simulink model "run_sim_paper_scenario"  (R2020a)
settings: Solver=ode4  StartTime=0.0  StopTime=30.0  FixedStep=0.01  RelTol=1e-3
values from neighbouring files (symbols this model uses):
  alfa_theta = 20    [init_sim_paper_scenario.m]
  alfa_theta_obs = 100    [init_sim_paper_scenario.m]
  beta1 = 1.2    [init_sim_paper_scenario.m]
  beta2 = 0.8    [init_sim_paper_scenario.m]
  beta_Phi_1 = pp0 * cal_frac_squ( 3, p_p0_plus_1, q_p0_plus_1 )                          * cal_frac_squ( eps_s_bar / pi, p_p0_min_2, q_p0_min_2 )                          / ( 2 * ( 2 * pp0 - 1 ) * tanh( gamma0 * ( eps_s_bar / pi ) / 2 ) )                          - ( cal_frac_squ( 3, p_p0_plus_1, q_p0_plus_1 ) * gamma0 / ( 4 * ( 2 * pp0 -1 ) ) )                          * cal_frac_squ( eps_s_bar / pi, p_p0_min_ ...(+136 chars)    [init_sim_paper_scenario.m]
  beta_Phi_2 = ( 1 - pp0 ) * cal_frac_squ( 3, p_p0_plus_1, q_p0_plus_1 )                          / ( 2 * ( 1 - 2 * pp0 ) * cal_frac_squ( eps_s_bar / pi, p_p0_0, q_p0_0 ) * tanh( gamma0 * ( eps_s_bar / pi ) / 2 ) )                          - ( cal_frac_squ( 3, p_p0_plus_1, q_p0_plus_1 ) * gamma0 / ( 4 * ( 1 - 2 * pp0 ) ) )                          * cal_frac_squ( eps_s_bar / pi, p_1_min_p0, q_1_min_p0 )          ...(+112 chars)    [init_sim_paper_scenario.m]
  c1_diff_sigma_bar_v = diag([25; 30; 20])    [init_sim_paper_scenario.m]
  c1_diff_sigma_bar_w = diag([12; 12; 12])    [init_sim_paper_scenario.m]
  c1_diff_ui = diag([25; 30; 20])    [init_sim_paper_scenario.m]
  c1v = diag([5.8; 6.5; 6.5])    [init_sim_paper_scenario.m]
  c2_diff_sigma_bar_v = diag([50; 50; 10])    [init_sim_paper_scenario.m]
  c2_diff_sigma_bar_w = diag([12; 12; 12])    [init_sim_paper_scenario.m]
  c2_diff_ui = diag([50; 50; 10])    [init_sim_paper_scenario.m]
  c2v = diag([5.8; 6.5; 6.5])    [init_sim_paper_scenario.m]
  c3_diff_sigma_bar_v = diag([15; 15; 10])    [init_sim_paper_scenario.m]
  c3_diff_sigma_bar_w = diag([15; 15; 15])    [init_sim_paper_scenario.m]
  c3_diff_ui = diag([15; 15; 10])    [init_sim_paper_scenario.m]
  c3v = diag([4.8; 6.4; 6.0])    [init_sim_paper_scenario.m]
  c_w_1 = diag( [20; 15; 15] )    [init_sim_paper_scenario.m]
  c_w_2 = diag( [20; 15; 15] )    [init_sim_paper_scenario.m]
  c_w_3 = diag( [2; 2; 2] )    [init_sim_paper_scenario.m]
  cS0 = diag( [4.5; 4.5; 4.5] )    [init_sim_paper_scenario.m]
  delta_p_i_0 = zeros(3, NF)    [init_sim_paper_scenario.m]
  delta_v_i_0 = zeros(3, NF)    [init_sim_paper_scenario.m]
  dp_aa_t = 0.2 * ones(3, 5) + ( 1.0 - 0.2 ) * rand(3, 5)    [init_sim_paper_scenario.m]
  dp_ff_t = [ 0.4 * ones(1, 5) + ( 1.0 - 0.4 ) * rand(1, 5);                      0.4 * ones(1, 5) + ( 1.0 - 0.4 ) * rand(1, 5);                      0.2 * ones(1, 5) + ( 0.6 - 0.2 ) * rand(1, 5) ]    [init_sim_paper_scenario.m]
  dp_phi_t = ( - pi / 2 ) * ones(3, 5) + ( pi / 2 - ( - pi / 2 ) ) * rand(3, 5)    [init_sim_paper_scenario.m]
  dw_aa_t = 0.2 * ones(3, 5) + ( 1.0 - 0.2 ) * rand(3, 5)    [init_sim_paper_scenario.m]
  dw_ff_t = [ 0.4 * ones(1, 5) + ( 1.0 - 0.4 ) * rand(1, 5);                      0.4 * ones(1, 5) + ( 1.0 - 0.4 ) * rand(1, 5);                      0.2 * ones(1, 5) + ( 0.6 - 0.2 ) * rand(1, 5) ]    [init_sim_paper_scenario.m]
  dw_phi_t = ( - pi / 2 ) * ones(3, 5) + ( pi / 2 - ( - pi / 2 ) ) * rand(3, 5)    [init_sim_paper_scenario.m]
  dwci_init = zeros(3,5)    [init_sim_paper_scenario.m]
  eps_s_bar_div_pi = eps_s_bar / pi    (= 0.03)    [init_sim_paper_scenario.m]
  etai_0 = zeros(3,5)    [init_sim_paper_scenario.m]
  gamma0 = 20    [init_sim_paper_scenario.m]
  h1w = diag([20.0; 20.0; 20.0])    [init_sim_paper_scenario.m]
  h2w = diag([30.0; 35.0; 35.0])    [init_sim_paper_scenario.m]
  h3w = diag([30.0; 25.0; 30.0])    [init_sim_paper_scenario.m]
  Ji = zeros(3,3,NF)    [init_sim_paper_scenario.m]
  k_J_0 = diag( [1; 1; 1] )    [init_sim_paper_scenario.m]
  kai_1_t = 0.02    [init_sim_paper_scenario.m]
  kai_3_t = 0.1    [init_sim_paper_scenario.m]
  kai_chi_1 = diag([6; 6; 6])    [init_sim_paper_scenario.m]
  kai_chi_2 = diag([6; 6; 6])    [init_sim_paper_scenario.m]
  kai_u_1 = diag([8; 8; 8])    [init_sim_paper_scenario.m]
  kai_u_2 = diag([8; 8; 8])    [init_sim_paper_scenario.m]
  ksii_0 = zeros(3,5)    [init_sim_paper_scenario.m]
  l1v = diag([20; 20; 20])    [init_sim_paper_scenario.m]
  l2v = diag([30; 30; 30])    [init_sim_paper_scenario.m]
  Lamd_diff_sigma_bar_v = 0.5    [init_sim_paper_scenario.m]
  Lamd_diff_sigma_bar_w = 0.8    [init_sim_paper_scenario.m]
  Lamd_diff_ui = 0.8    [init_sim_paper_scenario.m]
  mass_i = zeros(1,NF)    [init_sim_paper_scenario.m]
  Mii = diag([1;0;0;0;1])    [init_sim_paper_scenario.m]
  mu_c_theta = 100    [init_sim_paper_scenario.m]
  mu_d_w = 100    [init_sim_paper_scenario.m]
  pos0 = zeros(3, 1)    [init_sim_paper_scenario.m]
  pp0 = 8 / 11    (= 0.727272727273)    [init_sim_paper_scenario.m]    (also in plot_sim_paper_scenario.m = plot3( ksi0(1, kkt), ksi0(2, kkt), ksi0(3, kkt),            )
  PZ0 = P0(3)    [init_sim_paper_scenario.m]
  PZ1 = 10    [init_sim_paper_scenario.m]
  Qci_init = repmat([1;0;0;0],1,NF)    [init_sim_paper_scenario.m]
  R0 = 4    [init_sim_paper_scenario.m]
  R1 = 8    [init_sim_paper_scenario.m]
  Rci_init = zeros(3,3,NF)    [init_sim_paper_scenario.m]
  Ri_init = zeros(3,3,NF)    [init_sim_paper_scenario.m]
  Rx2 = 10    [init_sim_paper_scenario.m]
  Ry2 = 6    [init_sim_paper_scenario.m]
  Rz2 = 4    [init_sim_paper_scenario.m]
  T0 = 0    [init_sim_paper_scenario.m]
  T1 = tseq1    (= 10)    [init_sim_paper_scenario.m]
  T12 = tseq1 + tseq12    (= 20)    [init_sim_paper_scenario.m]
  T2 = tseq1 + tseq12 + tseq2    (= 30)    [init_sim_paper_scenario.m]
  theta0 = ( 2 / 5 ) * pi    (= 1.25663706144)    [init_sim_paper_scenario.m]
  thr_p_plus_1 = cal_frac_squ( 3, p_p0_plus_1, q_p0_plus_1 )    [init_sim_paper_scenario.m]
  ui_init = zeros(3,NF)    [init_sim_paper_scenario.m]
  vel0 = zeros(3, 1)    [init_sim_paper_scenario.m]
  wci_init = zeros(3,5)    [init_sim_paper_scenario.m]
  Wij = [0,0,1,0,0;              0,0,1,1,0;              1,0,0,0,1;              0,1,1,0,0;              0,0,1,0,0]    [init_sim_paper_scenario.m]
  X1 = 8    [init_sim_paper_scenario.m]
  X2 = 2    [init_sim_paper_scenario.m]
  X3 = 3    [init_sim_paper_scenario.m]
  Y1 = 10    [init_sim_paper_scenario.m]
  Y2 = 2    [init_sim_paper_scenario.m]
  Y3 = 4    [init_sim_paper_scenario.m]
  Z1 = 4    [init_sim_paper_scenario.m]
  Z2 = -6    [init_sim_paper_scenario.m]
  Z3 = 2    [init_sim_paper_scenario.m]
  zeta_diff_sigma_bar_v = 0.08    [init_sim_paper_scenario.m]
  zeta_diff_sigma_bar_w = 0.3    [init_sim_paper_scenario.m]
  zeta_diff_ui = 0.05    [init_sim_paper_scenario.m]
undefined symbols (not defined in the file or in its folder): cal_frac_squ, p_2_p0, p_alfav1, p_alfav2, p_alfaw1, p_alfaw2, p_beta1, p_beta2, p_beta_w_1, p_beta_w_2, p_dbeta1, p_dbeta2, p_gamma1_pos, p_gamma1_vel, p_gamma2_pos, p_gamma2_vel, p_p0_min_1, p_p0_plus_1, q_2_p0, q_alfav1, q_alfav2, q_alfaw1, q_alfaw2, q_beta1, q_beta2, q_beta_w_1, q_beta_w_2, q_dbeta1, q_dbeta2, q_gamma1_pos, q_gamma1_vel, q_gamma2_pos, q_gamma2_vel, q_p0_min_1, q_p0_plus_1, Qei_init, Qi_init, Rei_init, V_Phi_Rei_init, wei_init, wi_init
(part 1 of 10)
settings Model: Creator=zzy  LastModifiedBy=Hershey.A
settings DataIOCC: ReturnWorkspaceOutputs=off
settings DebuggingCC: ArithmeticOperatorsInVariantConditions=warning
settings SFSimCC: SimUseLocalCustomCode=off  CustomCodeUndefinedFunction=UseInterfaceOnly
settings RTWCC: RTWUseLocalCustomCode=off

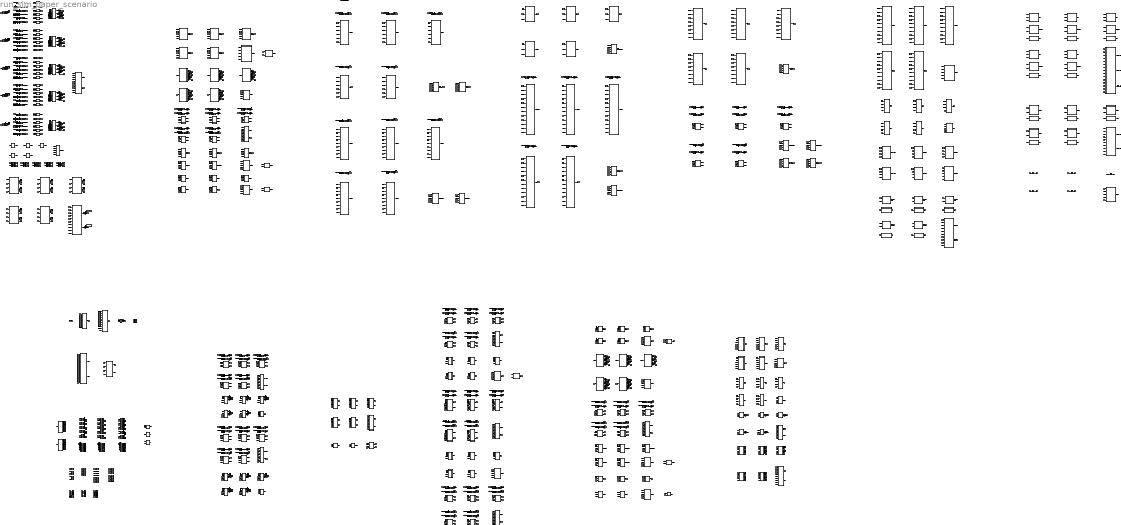
== system run_sim_paper_scenario ==
  Abs{,1..29} (30 alike) : Abs
  Add{,1..12,14,16..18,20..22,24..26,28..29} (25 alike) : Sum
  Add{13,15,19,23,27} (5 alike) : Sum  Inputs=+-
  Clock : Clock
  Constant : Constant  Value=T1
  Constant{1,4,9,19,24,149,154,159,164,169} (10 alike) : Constant  Value=q_beta1
  Constant{5,10,14,16,20,39,46,54,61,79,101,103,108,113,118,148,153,158,163,168} (20 alike) : Constant  Value=alfa_theta
  Constant{100,102,107,112,117} (5 alike) : Constant  Value=p_alfav1
  Constant{97,104,109,114,119} (5 alike) : Constant  Value=q_alfav1
  Constant{98,105,110,115,120} (5 alike) : Constant  Value=p_alfav2
  Constant{99,106,111,116,121} (5 alike) : Constant  Value=q_alfav2
  Constant{2,6,11,15,21,150,155,160,165,170} (10 alike) : Constant  Value=p_beta2
  Constant{3,7,12,17,22,151,156,161,166,171} (10 alike) : Constant  Value=q_beta2
  Constant{122,124,126,128,140} (5 alike) : Constant  Value=c1v
  Constant{123,125,127,139,141} (5 alike) : Constant  Value=c2v
  Constant129 : Constant  Value=R0
  Constant{8,13,18,23,63,147,152,157,162,167} (10 alike) : Constant  Value=p_beta1
  Constant130 : Constant  Value=R1
  Constant131 : Constant  Value=T0
  Constant132 : Constant  Value=Rz2
  Constant133 : Constant  Value=Ry2
  Constant134 : Constant  Value=Rx2
  Constant135 : Constant  Value=X1
  Constant136 : Constant  Value=X2
  Constant137 : Constant  Value=Y1
  Constant138 : Constant  Value=Y2
  Constant{92..96,142..146} (10 alike) : Constant  Value=c3v
  Constant{172,174,176,178,180} (5 alike) : Constant  Value=kai_u_1
  Constant{173,175,177,179,181} (5 alike) : Constant  Value=kai_u_2
  Constant{182..183,189,199,202,205,209,212,219,252} (10 alike) : Constant  Value=l2v
  Constant{184..186,193..196,198,283..284} (10 alike) : Constant  Value=alfa_theta_obs
  Constant{187,190,197,200,203,206,210,213,230,263} (10 alike) : Constant  Value=l1v
  Constant188 : Constant  Value=delta_p_i_0(:,4)
  Constant191 : Constant  Value=mass_i
  Constant192 : Constant  Value=delta_p_i_0(:,5)
  Constant201 : Constant  Value=delta_v_i_0(:,1)
  Constant204 : Constant  Value=delta_v_i_0(:,2)
  Constant207 : Constant  Value=delta_v_i_0(:,3)
  Constant208 : Constant  Value=delta_p_i_0(:,1)
  Constant211 : Constant  Value=delta_v_i_0(:,4)
  Constant214 : Constant  Value=delta_v_i_0(:,5)
  Constant{215,220,270,275,279} (5 alike) : Constant  Value=p_gamma1_pos
  Constant{216,267,271,276,280} (5 alike) : Constant  Value=q_gamma1_pos
  Constant{217,268,272,277,281} (5 alike) : Constant  Value=p_gamma2_pos
  Constant{218,269,273,278,282} (5 alike) : Constant  Value=q_gamma2_pos
  Constant221 : Constant  Value=Z1
  Constant222 : Constant  Value=Z2
  Constant{223,227,232,236,240} (5 alike) : Constant  Value=Wij
  Constant{224,228,233,237,242} (5 alike) : Constant  Value=Mii
  Constant225 : Constant  Value=theta0
  Constant226 : Constant  Value=Z3
  Constant229 : Constant  Value=Y3
  Constant231 : Constant  Value=kai_1_t
  Constant234 : Constant  Value=X3
  Constant235 : Constant  Value=kai_3_t
  Constant238 : Constant  Value=T1
  Constant239 : Constant  Value=T12
  Constant241 : Constant  Value=delta_p_i_0(:,2)
  Constant{243,286,289,292,295} (5 alike) : Constant  Value=dp_phi_t
  Constant{244,287,290,293,296} (5 alike) : Constant  Value=dp_ff_t
  Constant{245,249,254,258,262} (5 alike) : Constant  Value=p_gamma1_vel
  Constant{246,250,255,259,264} (5 alike) : Constant  Value=q_gamma1_vel
  Constant{247,251,256,260,265} (5 alike) : Constant  Value=p_gamma2_vel
  Constant{248,253,257,261,266} (5 alike) : Constant  Value=q_gamma2_vel
  Constant{25,27,29,31,33,82,84,86,88,90} (10 alike) : Constant  Value=kai_chi_2
  Constant{26,28,30,32,34,83,85,87,89,91} (10 alike) : Constant  Value=kai_chi_1
  Constant274 : Constant  Value=delta_p_i_0(:,3)
  Constant{285,288,291,294,297} (5 alike) : Constant  Value=dp_aa_t
  Constant{298,331,362,619,639} (5 alike) : Constant  Value=0
  Constant{299,411,488,556,621} (5 alike) : Constant  Value=p_p0_plus_1
  Constant{300,355,433,510,521} (5 alike) : Constant  Value=p_2_p0
  Constant{301,306,308,310,316,321,324,326,343,347,352,354,357,363,590,593,598,601,603,620,624,629,631,634,640} (25 alike) : Constant
  Constant{302,309,312..313,317,325,327..328,345..346,348,356,358..359,364..365,591..592,594,602,615..616,622..623,625,633,635..636,641..642} (30 alike) : Constant  Value=3
  Constant{303,314,318,329,349,360,595,617,626,637} (10 alike) : Constant  Value=2
  Constant{304,319,350,596,627} (5 alike) : Constant  Value=c1_diff_ui
  Constant{305,320,351,597,628} (5 alike) : Constant  Value=c2_diff_ui
  Constant{307,323,353,600,630} (5 alike) : Constant  Value=c3_diff_ui
  Constant{311,366,444,522,577} (5 alike) : Constant  Value=q_2_p0
  Constant{315,330,361,618,638} (5 alike) : Constant  Value=Lamd_diff_ui
  Constant{322,377,455,483,485,487,490,492,533,588,609,611..614} (15 alike) : Constant  Value=cS0
  Constant{332,335,337,339,341} (5 alike) : Constant  Value=p_p0_min_1
  Constant{333,388,393,461,466,468,474,481,544..545,578,583,589,599,607} (15 alike) : Constant  Value=gamma0
  Constant{334,336,338,340,342} (5 alike) : Constant  Value=q_p0_min_1
  Constant{344,392,398..399,467,473,477,480,547,555,575,581,586,605,610} (15 alike) : Constant  Value=thr_p_plus_1
  Constant{35,42,49,57,75} (5 alike) : Constant  Value=q_dbeta1
  Constant{36,43,50,58,76} (5 alike) : Constant  Value=p_dbeta2
  Constant{367..376,378..382} (15 alike) : Constant  Value=zeta_diff_ui
  Constant{37,44,52,59,77} (5 alike) : Constant  Value=q_dbeta2
  Constant{38,45,53,60,78} (5 alike) : Constant  Value=p_dbeta1
  Constant{383..387,401,413,437,447,450..452,454,457,459,484,486,489,491,493,526,530,535,539,543} (25 alike) : Constant  Value=Ji
  Constant{389,395,463,470,476} (5 alike) : Constant  Value=pp0
  Constant{390,396,464,471,478,571,579,584,604,608} (10 alike) : Constant  Value=beta_Phi_1
  Constant{391,397,465,472,479,548..549,574,580,585} (10 alike) : Constant  Value=beta_Phi_2
  Constant{394,462,469,475,482,546,576,582,587,606} (10 alike) : Constant  Value=eps_s_bar_div_pi
  Constant{40,47,55,62,80} (5 alike) : Constant  Value=beta1
  Constant{400,425,445..446,448..449,453,456,458,460} (10 alike) : Constant  Value=h3w
  Constant{402,404,409,417,423} (5 alike) : Constant  Value=p_alfaw1
  Constant{403,405,412,418,424} (5 alike) : Constant  Value=mu_d_w
  Constant{406,414,419,426,429} (5 alike) : Constant  Value=q_alfaw1
  Constant{407,415,420,427,430} (5 alike) : Constant  Value=p_alfaw2
  Constant{408,416,421,428,431} (5 alike) : Constant  Value=q_alfaw2
  Constant{41,48,56,74,81} (5 alike) : Constant  Value=beta2
  Constant{410,422,499,560,632} (5 alike) : Constant  Value=q_p0_plus_1
  Constant{432,435,438,440,442} (5 alike) : Constant  Value=h1w
  Constant{434,436,439,441,443} (5 alike) : Constant  Value=h2w
  Constant{494,500,505,511,516} (5 alike) : Constant  Value=p_beta_w_1
  Constant{495,501,506,512,517} (5 alike) : Constant  Value=q_beta_w_1
  Constant{496,502,507,513,518} (5 alike) : Constant  Value=p_beta_w_2
  Constant{497,503,508,514,519} (5 alike) : Constant  Value=q_beta_w_2
  Constant{498,504,509,515,520} (5 alike) : Constant  Value=mu_c_theta
  Constant51 : Constant  Value=Qci_init
  Constant{523,527,531,536,540} (5 alike) : Constant  Value=c_w_1
  Constant{524,528,532,537,541} (5 alike) : Constant  Value=c_w_2
  Constant{525,529,534,538,542} (5 alike) : Constant  Value=c_w_3
  Constant{550..554} (5 alike) : Constant  Value=k_J_0
  Constant{557,561,564,567,570} (5 alike) : Constant  Value=dw_aa_t
  Constant{558,562,565,568,572} (5 alike) : Constant  Value=dw_ff_t
  Constant{559,563,566,569,573} (5 alike) : Constant  Value=dw_phi_t
  Constant64 : Constant  Value=T2
  Constant65 : Constant  Value=R0
  Constant66 : Constant  Value=R1
  Constant67 : Constant  Value=Rx2
  Constant68 : Constant  Value=Ry2
  Constant69 : Constant  Value=Rz2
  Constant70 : Constant  Value=T2
  Constant71 : Constant  Value=T1
  Constant72 : Constant  Value=PZ0
  Constant73 : Constant  Value=PZ1
  Demux{,1..141} (142 alike) : Demux  Outputs=3
  Display{1..5,7..21,26..63,69..172} (162 alike) : Display
  Integrator{1..15,46..50} (20 alike) : Integrator  InitialCondition=zeros(3,1)
  Integrator17 : Integrator  InitialCondition=V_Phi_Rei_init(:,2)
  Integrator19 : Integrator  InitialCondition=V_Phi_Rei_init(:,3)
  Integrator20 : Integrator  InitialCondition=V_Phi_Rei_init(:,1)
  Integrator21 : Integrator  InitialCondition=wi_init(:,1)
  Integrator22 : Integrator  InitialCondition=wi_init(:,2)
  Integrator23 : Integrator  InitialCondition=wi_init(:,3)
  Integrator24 : Integrator  InitialCondition=wi_init(:,4)
  Integrator25 : Integrator  InitialCondition=wi_init(:,5)
  Integrator26 : Integrator  InitialCondition=Qi_init(:,1)
  Integrator27 : Integrator  InitialCondition=Qi_init(:,2)
  Integrator28 : Integrator  InitialCondition=Qi_init(:,3)
  Integrator29 : Integrator  InitialCondition=Qi_init(:,4)
  Integrator30 : Integrator  InitialCondition=Qi_init(:,5)
  Integrator31 : Integrator  InitialCondition=Qei_init(:,1)
  Integrator32 : Integrator  InitialCondition=Qei_init(:,2)
  Integrator33 : Integrator  InitialCondition=Qei_init(:,3)
  Integrator34 : Integrator  InitialCondition=Qei_init(:,4)
  Integrator35 : Integrator  InitialCondition=Qei_init(:,5)
  Integrator42 : Integrator  InitialCondition=V_Phi_Rei_init(:,4)
  Integrator44 : Integrator  InitialCondition=V_Phi_Rei_init(:,5)
  Interpreted MATLAB Function{,1..124} (125 alike) : MATLABFcn  MATLABFcn=cal_frac_squ(u(1:3),u(4),u(5))
  Memory : Memory  InitialCondition=ui_init
  Memory1 : Memory  InitialCondition=etai_0
  Memory{9..11,13,18..25} (12 alike) : Memory  InitialCondition=zeros(3,5)
  Memory12 : Memory  InitialCondition=V_Phi_Rei_init
  Memory14 : Memory  InitialCondition=wci_init
  Memory15 : Memory  InitialCondition=dwci_init
  Memory16 : Memory  InitialCondition=Qci_init
  Memory17 : Memory  InitialCondition=Rci_init
  Memory2 : Memory  InitialCondition=ksii_0
  Memory3 : Memory  InitialCondition=Qi_init
  Memory4 : Memory  InitialCondition=Ri_init
  Memory5 : Memory  InitialCondition=wi_init
  Memory6 : Memory  InitialCondition=wei_init
  Memory7 : Memory  InitialCondition=Qei_init
  Memory8 : Memory  InitialCondition=Rei_init
  Mux{1..40,109..118,120..129,136..170,180,187..215} (125 alike) : Mux  Inputs=3
  Mux{41..108,119,130..135,171..179,181..186} (90 alike) : Mux  Inputs=2
  Product{,1..9} (10 alike) : Product
  Qei dynam agent 1 : MATLAB Function  TreatAsAtomicUnit=on
  Qei dynam agent 2 : MATLAB Function  TreatAsAtomicUnit=on
  Qei dynam agent 3 : MATLAB Function  TreatAsAtomicUnit=on
  Qei dynam agent 4 : MATLAB Function  TreatAsAtomicUnit=on
  Qei dynam agent 5 : MATLAB Function  TreatAsAtomicUnit=on
  Qi dynam agent 1 : MATLAB Function  TreatAsAtomicUnit=on
  Qi dynam agent 2 : MATLAB Function  TreatAsAtomicUnit=on
  Qi dynam agent 3 : MATLAB Function  TreatAsAtomicUnit=on
  Qi dynam agent 4 : MATLAB Function  TreatAsAtomicUnit=on
  Qi dynam agent 5 : MATLAB Function  TreatAsAtomicUnit=on
  Scope{1..2,13..15} (5 alike) : Scope  NumInputPorts=3
  Step : Step  Time=T1+0.01  SampleTime=0
  To Workspace : ToWorkspace  VariableName=eta_d_est_vec  SampleTime=-1
  To Workspace1 : ToWorkspace  VariableName=dp_hat_vec  SampleTime=-1
  To Workspace10 : ToWorkspace  VariableName=eta_track_err_vec  SampleTime=-1
  To Workspace11 : ToWorkspace  VariableName=sigma_bar_v_hat_vec  SampleTime=-1
  To Workspace12 : ToWorkspace  VariableName=sigma_bar_v_vec  SampleTime=-1
  To Workspace13 : ToWorkspace  VariableName=sigma_bar_v_tilt_vec  SampleTime=-1
  To Workspace14 : ToWorkspace  VariableName=ui_vec  SampleTime=-1
  To Workspace15 : ToWorkspace  VariableName=chi_vec  SampleTime=-1
  To Workspace16 : ToWorkspace  VariableName=phi_vec  SampleTime=-1
  To Workspace17 : ToWorkspace  VariableName=ksi_est_err  SampleTime=-1
  To Workspace18 : ToWorkspace  VariableName=ksi_d_est_vec  SampleTime=-1
  To Workspace19 : ToWorkspace  VariableName=sigma_v_vec  SampleTime=-1
  To Workspace2 : ToWorkspace  VariableName=dp_vec  SampleTime=-1
  To Workspace20 : ToWorkspace  VariableName=delta_ksi_vec  SampleTime=-1
  To Workspace21 : ToWorkspace  VariableName=delta_eta_vec  SampleTime=-1
  To Workspace22 : ToWorkspace  VariableName=eta_est_err  SampleTime=-1
  To Workspace23 : ToWorkspace  VariableName=wci  SampleTime=-1
  To Workspace24 : ToWorkspace  VariableName=V_Phi_Rei  SampleTime=-1
  To Workspace25 : ToWorkspace  VariableName=dwi_tilt  SampleTime=-1
  To Workspace26 : ToWorkspace  VariableName=Qci  SampleTime=-1
  To Workspace27 : ToWorkspace  VariableName=sigma_bar_w_hat  SampleTime=-1
  To Workspace28 : ToWorkspace  VariableName=wei  SampleTime=-1
  To Workspace29 : ToWorkspace  VariableName=sigma_w  SampleTime=-1
  To Workspace3 : ToWorkspace  VariableName=u0  SampleTime=-1
  To Workspace30 : ToWorkspace  VariableName=sigma_bar_w  SampleTime=-1
  To Workspace31 : ToWorkspace  VariableName=Phi_psi_e  SampleTime=-1
  To Workspace32 : ToWorkspace  VariableName=Phi_bar_psi_e  SampleTime=-1
  To Workspace33 : ToWorkspace  VariableName=Qei  SampleTime=-1
  To Workspace34 : ToWorkspace  VariableName=wi  SampleTime=-1
  To Workspace35 : ToWorkspace  VariableName=Qi  SampleTime=-1
  To Workspace36 : ToWorkspace  VariableName=S_bar  SampleTime=-1
  To Workspace37 : ToWorkspace  VariableName=Si  SampleTime=-1
  To Workspace38 : ToWorkspace  VariableName=dwi  SampleTime=-1
  To Workspace39 : ToWorkspace  VariableName=dwi_hat  SampleTime=-1
  To Workspace4 : ToWorkspace  VariableName=eta0  SampleTime=-1
  To Workspace5 : ToWorkspace  VariableName=ksi0  SampleTime=-1
  To Workspace6 : ToWorkspace  VariableName=dp_tilt_vec  SampleTime=-1
  To Workspace7 : ToWorkspace  VariableName=eta_i_vec  SampleTime=-1
  To Workspace8 : ToWorkspace  VariableName=ksi_i_vec  SampleTime=-1
  To Workspace9 : ToWorkspace  VariableName=ksi_track_err_vec  SampleTime=-1
  cal Fi_S agent 1 : MATLAB Function  TreatAsAtomicUnit=on
  cal Fi_S agent 2 : MATLAB Function  TreatAsAtomicUnit=on
  cal Fi_S agent 3 : MATLAB Function  TreatAsAtomicUnit=on
  cal Fi_S agent 4 : MATLAB Function  TreatAsAtomicUnit=on
  cal Fi_S agent 5 : MATLAB Function  TreatAsAtomicUnit=on
  cal Phi_bar_psi_e agent 1 : MATLAB Function  TreatAsAtomicUnit=on
  cal Phi_bar_psi_e agent 2 : MATLAB Function  TreatAsAtomicUnit=on
  cal Phi_bar_psi_e agent 3 : MATLAB Function  TreatAsAtomicUnit=on
  cal Phi_bar_psi_e agent 4 : MATLAB Function  TreatAsAtomicUnit=on
  cal Phi_bar_psi_e agent 5 : MATLAB Function  TreatAsAtomicUnit=on
  cal Phi_psi_e agent 1 : MATLAB Function  TreatAsAtomicUnit=on
  cal Phi_psi_e agent 2 : MATLAB Function  TreatAsAtomicUnit=on
  cal Phi_psi_e agent 3 : MATLAB Function  TreatAsAtomicUnit=on
  cal Phi_psi_e agent 4 : MATLAB Function  TreatAsAtomicUnit=on
  cal Phi_psi_e agent 5 : MATLAB Function  TreatAsAtomicUnit=on
  cal Qci agent 1 : MATLAB Function  TreatAsAtomicUnit=on
  cal Qci agent 2 : MATLAB Function  TreatAsAtomicUnit=on
  cal Qci agent 3 : MATLAB Function  TreatAsAtomicUnit=on
  cal Qci agent 4 : MATLAB Function  TreatAsAtomicUnit=on
  cal Qci agent 5 : MATLAB Function  TreatAsAtomicUnit=on
  cal Rci agent 1 : MATLAB Function  TreatAsAtomicUnit=on
  cal Rci agent 2 : MATLAB Function  TreatAsAtomicUnit=on
  cal Rci agent 3 : MATLAB Function  TreatAsAtomicUnit=on
  cal Rci agent 4 : MATLAB Function  TreatAsAtomicUnit=on
  cal Rci agent 5 : MATLAB Function  TreatAsAtomicUnit=on
  cal Rci from ui : MATLAB Function  TreatAsAtomicUnit=on
  cal Rei : MATLAB Function  TreatAsAtomicUnit=on
  cal Rei agent 1 : MATLAB Function  TreatAsAtomicUnit=on
  cal Rei agent 2 : MATLAB Function  TreatAsAtomicUnit=on
  cal Rei agent 3 : MATLAB Function  TreatAsAtomicUnit=on
  cal Rei agent 4 : MATLAB Function  TreatAsAtomicUnit=on
  cal Rei agent 5 : MATLAB Function  TreatAsAtomicUnit=on
  cal Ri : MATLAB Function  TreatAsAtomicUnit=on
  cal Ri agent 1 : MATLAB Function  TreatAsAtomicUnit=on
  cal Ri agent 2 : MATLAB Function  TreatAsAtomicUnit=on
  cal Ri agent 3 : MATLAB Function  TreatAsAtomicUnit=on
  cal Ri agent 4 : MATLAB Function  TreatAsAtomicUnit=on
  cal Ri agent 5 : MATLAB Function  TreatAsAtomicUnit=on
  cal S_bar agent 1 : MATLAB Function  TreatAsAtomicUnit=on
  cal S_bar agent 2 : MATLAB Function  TreatAsAtomicUnit=on
  cal S_bar agent 3 : MATLAB Function  TreatAsAtomicUnit=on
  cal S_bar agent 4 : MATLAB Function  TreatAsAtomicUnit=on
  cal S_bar agent 5 : MATLAB Function  TreatAsAtomicUnit=on
  cal Si agent 1 : MATLAB Function  TreatAsAtomicUnit=on
  cal Si agent 2 : MATLAB Function  TreatAsAtomicUnit=on
  cal Si agent 3 : MATLAB Function  TreatAsAtomicUnit=on
  cal Si agent 4 : MATLAB Function  TreatAsAtomicUnit=on
  cal Si agent 5 : MATLAB Function  TreatAsAtomicUnit=on
  cal abs 1 : MATLAB Function  TreatAsAtomicUnit=on
  cal abs 10 : MATLAB Function  TreatAsAtomicUnit=on
  cal abs 11 : MATLAB Function  TreatAsAtomicUnit=on
  cal abs 12 : MATLAB Function  TreatAsAtomicUnit=on
  cal abs 13 : MATLAB Function  TreatAsAtomicUnit=on
  cal abs 14 : MATLAB Function  TreatAsAtomicUnit=on
  cal abs 15 : MATLAB Function  TreatAsAtomicUnit=on
  cal abs 16 : MATLAB Function  TreatAsAtomicUnit=on
  cal abs 17 : MATLAB Function  TreatAsAtomicUnit=on
  cal abs 18 : MATLAB Function  TreatAsAtomicUnit=on
  cal abs 19 : MATLAB Function  TreatAsAtomicUnit=on
  cal abs 2 : MATLAB Function  TreatAsAtomicUnit=on
  cal abs 20 : MATLAB Function  TreatAsAtomicUnit=on
  cal abs 21 : MATLAB Function  TreatAsAtomicUnit=on
  cal abs 22 : MATLAB Function  TreatAsAtomicUnit=on
  cal abs 23 : MATLAB Function  TreatAsAtomicUnit=on
  cal abs 24 : MATLAB Function  TreatAsAtomicUnit=on
  cal abs 25 : MATLAB Function  TreatAsAtomicUnit=on
  cal abs 26 : MATLAB Function  TreatAsAtomicUnit=on
  cal abs 27 : MATLAB Function  TreatAsAtomicUnit=on
  cal abs 28 : MATLAB Function  TreatAsAtomicUnit=on
  cal abs 29 : MATLAB Function  TreatAsAtomicUnit=on
  cal abs 3 : MATLAB Function  TreatAsAtomicUnit=on
  cal abs 30 : MATLAB Function  TreatAsAtomicUnit=on
  cal abs 31 : MATLAB Function  TreatAsAtomicUnit=on
  cal abs 32 : MATLAB Function  TreatAsAtomicUnit=on
  cal abs 33 : MATLAB Function  TreatAsAtomicUnit=on
  cal abs 34 : MATLAB Function  TreatAsAtomicUnit=on
  cal abs 35 : MATLAB Function  TreatAsAtomicUnit=on
  cal abs 36 : MATLAB Function  TreatAsAtomicUnit=on
  cal abs 37 : MATLAB Function  TreatAsAtomicUnit=on
  cal abs 38 : MATLAB Function  TreatAsAtomicUnit=on
  cal abs 39 : MATLAB Function  TreatAsAtomicUnit=on
  cal abs 4 : MATLAB Function  TreatAsAtomicUnit=on
  cal abs 40 : MATLAB Function  TreatAsAtomicUnit=on
  cal abs 41 : MATLAB Function  TreatAsAtomicUnit=on
  cal abs 42 : MATLAB Function  TreatAsAtomicUnit=on
  cal abs 43 : MATLAB Function  TreatAsAtomicUnit=on
  cal abs 44 : MATLAB Function  TreatAsAtomicUnit=on
  cal abs 45 : MATLAB Function  TreatAsAtomicUnit=on
  cal abs 46 : MATLAB Function  TreatAsAtomicUnit=on
  cal abs 47 : MATLAB Function  TreatAsAtomicUnit=on
  cal abs 48 : MATLAB Function  TreatAsAtomicUnit=on
  cal abs 49 : MATLAB Function  TreatAsAtomicUnit=on
  cal abs 5 : MATLAB Function  TreatAsAtomicUnit=on
  cal abs 50 : MATLAB Function  TreatAsAtomicUnit=on
  cal abs 51 : MATLAB Function  TreatAsAtomicUnit=on
  cal abs 52 : MATLAB Function  TreatAsAtomicUnit=on
  cal abs 53 : MATLAB Function  TreatAsAtomicUnit=on
  cal abs 54 : MATLAB Function  TreatAsAtomicUnit=on
  cal abs 55 : MATLAB Function  TreatAsAtomicUnit=on
  cal abs 56 : MATLAB Function  TreatAsAtomicUnit=on
  cal abs 57 : MATLAB Function  TreatAsAtomicUnit=on
  cal abs 58 : MATLAB Function  TreatAsAtomicUnit=on
  cal abs 59 : MATLAB Function  TreatAsAtomicUnit=on
  cal abs 6 : MATLAB Function  TreatAsAtomicUnit=on
  cal abs 60 : MATLAB Function  TreatAsAtomicUnit=on
  cal abs 61 : MATLAB Function  TreatAsAtomicUnit=on
  cal abs 62 : MATLAB Function  TreatAsAtomicUnit=on
  cal abs 63 : MATLAB Function  TreatAsAtomicUnit=on
  cal abs 64 : MATLAB Function  TreatAsAtomicUnit=on
  cal abs 65 : MATLAB Function  TreatAsAtomicUnit=on
  cal abs 66 : MATLAB Function  TreatAsAtomicUnit=on
  cal abs 67 : MATLAB Function  TreatAsAtomicUnit=on
  cal abs 68 : MATLAB Function  TreatAsAtomicUnit=on
  cal abs 69 : MATLAB Function  TreatAsAtomicUnit=on
  cal abs 7 : MATLAB Function  TreatAsAtomicUnit=on
  cal abs 70 : MATLAB Function  TreatAsAtomicUnit=on
  cal abs 71 : MATLAB Function  TreatAsAtomicUnit=on
  cal abs 72 : MATLAB Function  TreatAsAtomicUnit=on
  cal abs 73 : MATLAB Function  TreatAsAtomicUnit=on
  cal abs 74 : MATLAB Function  TreatAsAtomicUnit=on
  cal abs 75 : MATLAB Function  TreatAsAtomicUnit=on
  cal abs 76 : MATLAB Function  TreatAsAtomicUnit=on
  cal abs 77 : MATLAB Function  TreatAsAtomicUnit=on
  cal abs 78 : MATLAB Function  TreatAsAtomicUnit=on
  cal abs 79 : MATLAB Function  TreatAsAtomicUnit=on
  cal abs 8 : MATLAB Function  TreatAsAtomicUnit=on
  cal abs 80 : MATLAB Function  TreatAsAtomicUnit=on
  cal abs 81 : MATLAB Function  TreatAsAtomicUnit=on
  cal abs 82 : MATLAB Function  TreatAsAtomicUnit=on
  cal abs 83 : MATLAB Function  TreatAsAtomicUnit=on
  cal abs 84 : MATLAB Function  TreatAsAtomicUnit=on
  cal abs 85 : MATLAB Function  TreatAsAtomicUnit=on
  cal abs 86 : MATLAB Function  TreatAsAtomicUnit=on
  cal abs 87 : MATLAB Function  TreatAsAtomicUnit=on
  cal abs 88 : MATLAB Function  TreatAsAtomicUnit=on
  cal abs 89 : MATLAB Function  TreatAsAtomicUnit=on
  cal abs 9 : MATLAB Function  TreatAsAtomicUnit=on
  cal abs 90 : MATLAB Function  TreatAsAtomicUnit=on
  cal abs 91 : MATLAB Function  TreatAsAtomicUnit=on
  cal abs 92 : MATLAB Function  TreatAsAtomicUnit=on
  cal abs 93 : MATLAB Function  TreatAsAtomicUnit=on
  cal abs 94 : MATLAB Function  TreatAsAtomicUnit=on
  cal abs 95 : MATLAB Function  TreatAsAtomicUnit=on
  cal combine sigma_bar_v : MATLAB Function  TreatAsAtomicUnit=on
  cal combine sigma_bar_v_tilt : MATLAB Function  TreatAsAtomicUnit=on
  cal combine sigma_bar_w_tilt : MATLAB Function  TreatAsAtomicUnit=on
  cal d_sigma_w agent 1 : MATLAB Function  TreatAsAtomicUnit=on
  cal d_sigma_w agent 2 : MATLAB Function  TreatAsAtomicUnit=on
  cal d_sigma_w agent 3 : MATLAB Function  TreatAsAtomicUnit=on
  cal d_sigma_w agent 4 : MATLAB Function  TreatAsAtomicUnit=on
  cal d_sigma_w agent 5 : MATLAB Function  TreatAsAtomicUnit=on
  cal d_theta_err_ksi agent 1 : MATLAB Function  TreatAsAtomicUnit=on
  cal d_theta_err_ksi agent 2 : MATLAB Function  TreatAsAtomicUnit=on
  cal d_theta_err_ksi agent 3 : MATLAB Function  TreatAsAtomicUnit=on
  cal d_theta_err_ksi agent 4 : MATLAB Function  TreatAsAtomicUnit=on
  cal d_theta_err_ksi agent 5 : MATLAB Function  TreatAsAtomicUnit=on
  cal dchi agent 1 : MATLAB Function  TreatAsAtomicUnit=on
  cal dchi agent 2 : MATLAB Function  TreatAsAtomicUnit=on
  cal dchi agent 3 : MATLAB Function  TreatAsAtomicUnit=on
  cal dchi agent 4 : MATLAB Function  TreatAsAtomicUnit=on
  cal dchi agent 5 : MATLAB Function  TreatAsAtomicUnit=on
  cal differentiator d_sigma_bar_v_hat agent 1 : Subsystem
  cal differentiator d_sigma_bar_v_hat agent 2 : Subsystem
  cal differentiator d_sigma_bar_v_hat agent 3 : Subsystem
  cal differentiator d_sigma_bar_v_hat agent 4 : Subsystem
  cal differentiator d_sigma_bar_v_hat agent 5 : Subsystem
  cal differentiator d_sigma_bar_w_hat agent 1 : Subsystem
  cal differentiator d_sigma_bar_w_hat agent 2 : Subsystem
  cal differentiator d_sigma_bar_w_hat agent 3 : Subsystem
  cal differentiator d_sigma_bar_w_hat agent 4 : Subsystem
  cal differentiator d_sigma_bar_w_hat agent 5 : Subsystem
  cal disturbance observation error dp_tilt : MATLAB Function  TreatAsAtomicUnit=on
  cal divide pi : MATLAB Function  TreatAsAtomicUnit=on
  cal dp_hat agent 1 : MATLAB Function  TreatAsAtomicUnit=on
  cal dp_hat agent 2 : MATLAB Function  TreatAsAtomicUnit=on
  cal dp_hat agent 3 : MATLAB Function  TreatAsAtomicUnit=on
  cal dp_hat agent 4 : MATLAB Function  TreatAsAtomicUnit=on
  cal dp_hat agent 5 : MATLAB Function  TreatAsAtomicUnit=on
  cal duihat d2uihat by high-order differentiator node 1 : MATLAB Function  TreatAsAtomicUnit=on
  cal duihat d2uihat by high-order differentiator node 2 : MATLAB Function  TreatAsAtomicUnit=on
  cal duihat d2uihat by high-order differentiator node 3 : MATLAB Function  TreatAsAtomicUnit=on
  cal duihat d2uihat by high-order differentiator node 4 : MATLAB Function  TreatAsAtomicUnit=on
  cal duihat d2uihat by high-order differentiator node 5 : MATLAB Function  TreatAsAtomicUnit=on
  cal dw_hat agent 1 : MATLAB Function  TreatAsAtomicUnit=on
  cal dw_hat agent 2 : MATLAB Function  TreatAsAtomicUnit=on
  cal dw_hat agent 3 : MATLAB Function  TreatAsAtomicUnit=on
  cal dw_hat agent 4 : MATLAB Function  TreatAsAtomicUnit=on
  cal dw_hat agent 5 : MATLAB Function  TreatAsAtomicUnit=on
  cal error dw_tilt : MATLAB Function  TreatAsAtomicUnit=on
  cal formation tracking position and velocity errors : MATLAB Function  TreatAsAtomicUnit=on
  cal lumped observation error agent 1 : MATLAB Function  TreatAsAtomicUnit=on
  cal lumped observation error agent 2 : MATLAB Function  TreatAsAtomicUnit=on
  cal lumped observation error agent 3 : MATLAB Function  TreatAsAtomicUnit=on
  cal lumped observation error agent 4 : MATLAB Function  TreatAsAtomicUnit=on
  cal lumped observation error agent 5 : MATLAB Function  TreatAsAtomicUnit=on
  cal position estimate error : MATLAB Function  TreatAsAtomicUnit=on
  cal sig : MATLAB Function  TreatAsAtomicUnit=on
  cal sig1 : MATLAB Function  TreatAsAtomicUnit=on
  cal sig10 : MATLAB Function  TreatAsAtomicUnit=on
  cal sig11 : MATLAB Function  TreatAsAtomicUnit=on
  cal sig12 : MATLAB Function  TreatAsAtomicUnit=on
  cal sig13 : MATLAB Function  TreatAsAtomicUnit=on
  cal sig14 : MATLAB Function  TreatAsAtomicUnit=on
  cal sig15 : MATLAB Function  TreatAsAtomicUnit=on
  cal sig16 : MATLAB Function  TreatAsAtomicUnit=on
  cal sig17 : MATLAB Function  TreatAsAtomicUnit=on
  cal sig18 : MATLAB Function  TreatAsAtomicUnit=on
  cal sig19 : MATLAB Function  TreatAsAtomicUnit=on
  cal sig2 : MATLAB Function  TreatAsAtomicUnit=on
  cal sig20 : MATLAB Function  TreatAsAtomicUnit=on
  cal sig21 : MATLAB Function  TreatAsAtomicUnit=on
  cal sig22 : MATLAB Function  TreatAsAtomicUnit=on
  cal sig23 : MATLAB Function  TreatAsAtomicUnit=on
  cal sig24 : MATLAB Function  TreatAsAtomicUnit=on
  cal sig25 : MATLAB Function  TreatAsAtomicUnit=on
  cal sig26 : MATLAB Function  TreatAsAtomicUnit=on
  cal sig27 : MATLAB Function  TreatAsAtomicUnit=on
  cal sig28 : MATLAB Function  TreatAsAtomicUnit=on
  cal sig29 : MATLAB Function  TreatAsAtomicUnit=on
  cal sig3 : MATLAB Function  TreatAsAtomicUnit=on
  cal sig4 : MATLAB Function  TreatAsAtomicUnit=on
  cal sig5 : MATLAB Function  TreatAsAtomicUnit=on
  cal sig6 : MATLAB Function  TreatAsAtomicUnit=on
  cal sig7 : MATLAB Function  TreatAsAtomicUnit=on
  cal sig8 : MATLAB Function  TreatAsAtomicUnit=on
  cal sig9 : MATLAB Function  TreatAsAtomicUnit=on
  cal sigma_bar_v_hat agent 1 : MATLAB Function  TreatAsAtomicUnit=on
  cal sigma_bar_v_hat agent 2 : MATLAB Function  TreatAsAtomicUnit=on
  cal sigma_bar_v_hat agent 3 : MATLAB Function  TreatAsAtomicUnit=on
  cal sigma_bar_v_hat agent 4 : MATLAB Function  TreatAsAtomicUnit=on
  cal sigma_bar_v_hat agent 5 : MATLAB Function  TreatAsAtomicUnit=on
  cal sigma_bar_w_hat agent 1 : MATLAB Function  TreatAsAtomicUnit=on
  cal sigma_bar_w_hat agent 2 : MATLAB Function  TreatAsAtomicUnit=on
  cal sigma_bar_w_hat agent 3 : MATLAB Function  TreatAsAtomicUnit=on
  cal sigma_bar_w_hat agent 4 : MATLAB Function  TreatAsAtomicUnit=on
  cal sigma_bar_w_hat agent 5 : MATLAB Function  TreatAsAtomicUnit=on
  cal sigma_w_bar : MATLAB Function  TreatAsAtomicUnit=on
  cal taui agent 1 : MATLAB Function  TreatAsAtomicUnit=on
  cal taui agent 2 : MATLAB Function  TreatAsAtomicUnit=on
  cal taui agent 3 : MATLAB Function  TreatAsAtomicUnit=on
  cal taui agent 4 : MATLAB Function  TreatAsAtomicUnit=on
  cal taui agent 5 : MATLAB Function  TreatAsAtomicUnit=on
  cal theta_Si_beta_w agent 1 : MATLAB Function  TreatAsAtomicUnit=on
  cal theta_Si_beta_w agent 2 : MATLAB Function  TreatAsAtomicUnit=on
  cal theta_Si_beta_w agent 3 : MATLAB Function  TreatAsAtomicUnit=on
  cal theta_Si_beta_w agent 4 : MATLAB Function  TreatAsAtomicUnit=on
  cal theta_Si_beta_w agent 5 : MATLAB Function  TreatAsAtomicUnit=on
  cal theta_err_ksi agent 1 : MATLAB Function  TreatAsAtomicUnit=on
  cal theta_err_ksi agent 2 : MATLAB Function  TreatAsAtomicUnit=on
  cal theta_err_ksi agent 3 : MATLAB Function  TreatAsAtomicUnit=on
  cal theta_err_ksi agent 4 : MATLAB Function  TreatAsAtomicUnit=on
  cal theta_err_ksi agent 5 : MATLAB Function  TreatAsAtomicUnit=on
  cal theta_eta_est_err_tilt agent 1 : MATLAB Function  TreatAsAtomicUnit=on
  cal theta_eta_est_err_tilt agent 2 : MATLAB Function  TreatAsAtomicUnit=on
  cal theta_eta_est_err_tilt agent 3 : MATLAB Function  TreatAsAtomicUnit=on
  cal theta_eta_est_err_tilt agent 4 : MATLAB Function  TreatAsAtomicUnit=on
  cal theta_eta_est_err_tilt agent 5 : MATLAB Function  TreatAsAtomicUnit=on
  cal theta_ksi_est_err_tilt agent 1 : MATLAB Function  TreatAsAtomicUnit=on
  cal theta_ksi_est_err_tilt agent 2 : MATLAB Function  TreatAsAtomicUnit=on
  cal theta_ksi_est_err_tilt agent 3 : MATLAB Function  TreatAsAtomicUnit=on
  cal theta_ksi_est_err_tilt agent 4 : MATLAB Function  TreatAsAtomicUnit=on
  cal theta_ksi_est_err_tilt agent 5 : MATLAB Function  TreatAsAtomicUnit=on
  cal theta_phi agent 1 : MATLAB Function  TreatAsAtomicUnit=on
  cal theta_phi agent 2 : MATLAB Function  TreatAsAtomicUnit=on
  cal theta_phi agent 3 : MATLAB Function  TreatAsAtomicUnit=on
  cal theta_phi agent 4 : MATLAB Function  TreatAsAtomicUnit=on
  cal theta_phi agent 5 : MATLAB Function  TreatAsAtomicUnit=on
  cal theta_sigma_bar_v_tilt agent 1 : MATLAB Function  TreatAsAtomicUnit=on
  cal theta_sigma_bar_v_tilt agent 2 : MATLAB Function  TreatAsAtomicUnit=on
  cal theta_sigma_bar_v_tilt agent 3 : MATLAB Function  TreatAsAtomicUnit=on
  cal theta_sigma_bar_v_tilt agent 4 : MATLAB Function  TreatAsAtomicUnit=on
  cal theta_sigma_bar_v_tilt agent 5 : MATLAB Function  TreatAsAtomicUnit=on
  cal theta_sigma_bar_w_tilt agent 1 : MATLAB Function  TreatAsAtomicUnit=on
  cal theta_sigma_bar_w_tilt agent 2 : MATLAB Function  TreatAsAtomicUnit=on
  cal theta_sigma_bar_w_tilt agent 3 : MATLAB Function  TreatAsAtomicUnit=on
  cal theta_sigma_bar_w_tilt agent 4 : MATLAB Function  TreatAsAtomicUnit=on
  cal theta_sigma_bar_w_tilt agent 5 : MATLAB Function  TreatAsAtomicUnit=on
  cal ui agent 1 : MATLAB Function  TreatAsAtomicUnit=on
  cal ui agent 2 : MATLAB Function  TreatAsAtomicUnit=on
  cal ui agent 3 : MATLAB Function  TreatAsAtomicUnit=on
  cal ui agent 4 : MATLAB Function  TreatAsAtomicUnit=on
  cal ui agent 5 : MATLAB Function  TreatAsAtomicUnit=on
  cal velocity estimate error : MATLAB Function  TreatAsAtomicUnit=on
  cal virtual control sigma_v agent 1 : MATLAB Function  TreatAsAtomicUnit=on
  cal virtual control sigma_v agent 2 : MATLAB Function  TreatAsAtomicUnit=on
  cal virtual control sigma_v agent 3 : MATLAB Function  TreatAsAtomicUnit=on
  cal virtual control sigma_v agent 4 : MATLAB Function  TreatAsAtomicUnit=on
  cal virtual control sigma_v agent 5 : MATLAB Function  TreatAsAtomicUnit=on
  cal virtual velocity control error phi : MATLAB Function  TreatAsAtomicUnit=on
  cal wci dwci agent 1 : MATLAB Function  TreatAsAtomicUnit=on
  cal wci dwci agent 2 : MATLAB Function  TreatAsAtomicUnit=on
  cal wci dwci agent 3 : MATLAB Function  TreatAsAtomicUnit=on
  cal wci dwci agent 4 : MATLAB Function  TreatAsAtomicUnit=on
  cal wci dwci agent 5 : MATLAB Function  TreatAsAtomicUnit=on
  cal wei agent 1 : MATLAB Function  TreatAsAtomicUnit=on
  cal wei agent 2 : MATLAB Function  TreatAsAtomicUnit=on
  cal wei agent 3 : MATLAB Function  TreatAsAtomicUnit=on
  cal wei agent 4 : MATLAB Function  TreatAsAtomicUnit=on
  cal wei agent 5 : MATLAB Function  TreatAsAtomicUnit=on
  choose chi_1 : MATLAB Function  TreatAsAtomicUnit=on
  choose chi_2 : MATLAB Function  TreatAsAtomicUnit=on
  choose chi_3 : MATLAB Function  TreatAsAtomicUnit=on
  choose chi_4 : MATLAB Function  TreatAsAtomicUnit=on
  choose chi_5 : MATLAB Function  TreatAsAtomicUnit=on
  choose dp_1 : MATLAB Function  TreatAsAtomicUnit=on
  choose dp_2 : MATLAB Function  TreatAsAtomicUnit=on
  choose dp_3 : MATLAB Function  TreatAsAtomicUnit=on
  choose dp_4 : MATLAB Function  TreatAsAtomicUnit=on
  choose dp_5 : MATLAB Function  TreatAsAtomicUnit=on
  choose dp_hat_1 : MATLAB Function  TreatAsAtomicUnit=on
  choose dp_hat_2 : MATLAB Function  TreatAsAtomicUnit=on
  choose dp_hat_3 : MATLAB Function  TreatAsAtomicUnit=on
  choose dp_hat_4 : MATLAB Function  TreatAsAtomicUnit=on
  choose dp_hat_5 : MATLAB Function  TreatAsAtomicUnit=on
  choose dp_tilt_1 : MATLAB Function  TreatAsAtomicUnit=on
  choose dp_tilt_2 : MATLAB Function  TreatAsAtomicUnit=on
  choose dp_tilt_3 : MATLAB Function  TreatAsAtomicUnit=on
  choose dp_tilt_4 : MATLAB Function  TreatAsAtomicUnit=on
  choose dp_tilt_5 : MATLAB Function  TreatAsAtomicUnit=on
  choose err_eta_1 : MATLAB Function  TreatAsAtomicUnit=on
  choose err_eta_2 : MATLAB Function  TreatAsAtomicUnit=on
  choose err_eta_3 : MATLAB Function  TreatAsAtomicUnit=on
  choose err_eta_4 : MATLAB Function  TreatAsAtomicUnit=on
  choose err_eta_5 : MATLAB Function  TreatAsAtomicUnit=on
  choose eta_est_err_tilt 1 : MATLAB Function  TreatAsAtomicUnit=on
  choose eta_est_err_tilt 10 : MATLAB Function  TreatAsAtomicUnit=on
  choose eta_est_err_tilt 11 : MATLAB Function  TreatAsAtomicUnit=on
  choose eta_est_err_tilt 12 : MATLAB Function  TreatAsAtomicUnit=on
  choose eta_est_err_tilt 13 : MATLAB Function  TreatAsAtomicUnit=on
  choose eta_est_err_tilt 14 : MATLAB Function  TreatAsAtomicUnit=on
  choose eta_est_err_tilt 15 : MATLAB Function  TreatAsAtomicUnit=on
  choose eta_est_err_tilt 16 : MATLAB Function  TreatAsAtomicUnit=on
  choose eta_est_err_tilt 17 : MATLAB Function  TreatAsAtomicUnit=on
  choose eta_est_err_tilt 18 : MATLAB Function  TreatAsAtomicUnit=on
  choose eta_est_err_tilt 19 : MATLAB Function  TreatAsAtomicUnit=on
  choose eta_est_err_tilt 2 : MATLAB Function  TreatAsAtomicUnit=on
  choose eta_est_err_tilt 20 : MATLAB Function  TreatAsAtomicUnit=on
  choose eta_est_err_tilt 3 : MATLAB Function  TreatAsAtomicUnit=on
  choose eta_est_err_tilt 4 : MATLAB Function  TreatAsAtomicUnit=on
  choose eta_est_err_tilt 5 : MATLAB Function  TreatAsAtomicUnit=on
  choose eta_est_err_tilt 6 : MATLAB Function  TreatAsAtomicUnit=on
  choose eta_est_err_tilt 7 : MATLAB Function  TreatAsAtomicUnit=on
  choose eta_est_err_tilt 8 : MATLAB Function  TreatAsAtomicUnit=on
  choose eta_est_err_tilt 9 : MATLAB Function  TreatAsAtomicUnit=on
  choose ksi_est_err 1 : MATLAB Function  TreatAsAtomicUnit=on
  choose ksi_est_err 10 : MATLAB Function  TreatAsAtomicUnit=on
  choose ksi_est_err 11 : MATLAB Function  TreatAsAtomicUnit=on
  choose ksi_est_err 12 : MATLAB Function  TreatAsAtomicUnit=on
  choose ksi_est_err 13 : MATLAB Function  TreatAsAtomicUnit=on
  choose ksi_est_err 14 : MATLAB Function  TreatAsAtomicUnit=on
  choose ksi_est_err 15 : MATLAB Function  TreatAsAtomicUnit=on
  choose ksi_est_err 16 : MATLAB Function  TreatAsAtomicUnit=on
  choose ksi_est_err 17 : MATLAB Function  TreatAsAtomicUnit=on
  choose ksi_est_err 18 : MATLAB Function  TreatAsAtomicUnit=on
  choose ksi_est_err 19 : MATLAB Function  TreatAsAtomicUnit=on
  choose ksi_est_err 2 : MATLAB Function  TreatAsAtomicUnit=on
  choose ksi_est_err 20 : MATLAB Function  TreatAsAtomicUnit=on
  choose ksi_est_err 21 : MATLAB Function  TreatAsAtomicUnit=on
  choose ksi_est_err 22 : MATLAB Function  TreatAsAtomicUnit=on
  choose ksi_est_err 23 : MATLAB Function  TreatAsAtomicUnit=on
  choose ksi_est_err 24 : MATLAB Function  TreatAsAtomicUnit=on
  choose ksi_est_err 25 : MATLAB Function  TreatAsAtomicUnit=on
  choose ksi_est_err 26 : MATLAB Function  TreatAsAtomicUnit=on
  choose ksi_est_err 27 : MATLAB Function  TreatAsAtomicUnit=on
  choose ksi_est_err 28 : MATLAB Function  TreatAsAtomicUnit=on
  choose ksi_est_err 29 : MATLAB Function  TreatAsAtomicUnit=on
  choose ksi_est_err 3 : MATLAB Function  TreatAsAtomicUnit=on
  choose ksi_est_err 30 : MATLAB Function  TreatAsAtomicUnit=on
  choose ksi_est_err 31 : MATLAB Function  TreatAsAtomicUnit=on
  choose ksi_est_err 32 : MATLAB Function  TreatAsAtomicUnit=on
  choose ksi_est_err 33 : MATLAB Function  TreatAsAtomicUnit=on
  choose ksi_est_err 34 : MATLAB Function  TreatAsAtomicUnit=on
  choose ksi_est_err 35 : MATLAB Function  TreatAsAtomicUnit=on
  choose ksi_est_err 36 : MATLAB Function  TreatAsAtomicUnit=on
  choose ksi_est_err 37 : MATLAB Function  TreatAsAtomicUnit=on
  choose ksi_est_err 38 : MATLAB Function  TreatAsAtomicUnit=on
  choose ksi_est_err 39 : MATLAB Function  TreatAsAtomicUnit=on
  choose ksi_est_err 4 : MATLAB Function  TreatAsAtomicUnit=on
  choose ksi_est_err 40 : MATLAB Function  TreatAsAtomicUnit=on
  choose ksi_est_err 41 : MATLAB Function  TreatAsAtomicUnit=on
  choose ksi_est_err 42 : MATLAB Function  TreatAsAtomicUnit=on
  choose ksi_est_err 43 : MATLAB Function  TreatAsAtomicUnit=on
  choose ksi_est_err 44 : MATLAB Function  TreatAsAtomicUnit=on
  choose ksi_est_err 45 : MATLAB Function  TreatAsAtomicUnit=on
  choose ksi_est_err 46 : MATLAB Function  TreatAsAtomicUnit=on
  choose ksi_est_err 47 : MATLAB Function  TreatAsAtomicUnit=on
  choose ksi_est_err 48 : MATLAB Function  TreatAsAtomicUnit=on
  choose ksi_est_err 49 : MATLAB Function  TreatAsAtomicUnit=on
  choose ksi_est_err 5 : MATLAB Function  TreatAsAtomicUnit=on
  choose ksi_est_err 50 : MATLAB Function  TreatAsAtomicUnit=on
  choose ksi_est_err 51 : MATLAB Function  TreatAsAtomicUnit=on
  choose ksi_est_err 52 : MATLAB Function  TreatAsAtomicUnit=on
  choose ksi_est_err 53 : MATLAB Function  TreatAsAtomicUnit=on
  choose ksi_est_err 54 : MATLAB Function  TreatAsAtomicUnit=on
  choose ksi_est_err 55 : MATLAB Function  TreatAsAtomicUnit=on
  choose ksi_est_err 56 : MATLAB Function  TreatAsAtomicUnit=on
  choose ksi_est_err 57 : MATLAB Function  TreatAsAtomicUnit=on
  choose ksi_est_err 58 : MATLAB Function  TreatAsAtomicUnit=on
  choose ksi_est_err 59 : MATLAB Function  TreatAsAtomicUnit=on
  choose ksi_est_err 6 : MATLAB Function  TreatAsAtomicUnit=on
  choose ksi_est_err 60 : MATLAB Function  TreatAsAtomicUnit=on
  choose ksi_est_err 61 : MATLAB Function  TreatAsAtomicUnit=on
  choose ksi_est_err 62 : MATLAB Function  TreatAsAtomicUnit=on
  choose ksi_est_err 63 : MATLAB Function  TreatAsAtomicUnit=on
  choose ksi_est_err 64 : MATLAB Function  TreatAsAtomicUnit=on
  choose ksi_est_err 65 : MATLAB Function  TreatAsAtomicUnit=on
  choose ksi_est_err 66 : MATLAB Function  TreatAsAtomicUnit=on
  choose ksi_est_err 67 : MATLAB Function  TreatAsAtomicUnit=on
  choose ksi_est_err 68 : MATLAB Function  TreatAsAtomicUnit=on
  choose ksi_est_err 69 : MATLAB Function  TreatAsAtomicUnit=on
  choose ksi_est_err 7 : MATLAB Function  TreatAsAtomicUnit=on
  choose ksi_est_err 70 : MATLAB Function  TreatAsAtomicUnit=on
  choose ksi_est_err 71 : MATLAB Function  TreatAsAtomicUnit=on
  choose ksi_est_err 72 : MATLAB Function  TreatAsAtomicUnit=on
  choose ksi_est_err 73 : MATLAB Function  TreatAsAtomicUnit=on
  choose ksi_est_err 74 : MATLAB Function  TreatAsAtomicUnit=on
  choose ksi_est_err 75 : MATLAB Function  TreatAsAtomicUnit=on
  choose ksi_est_err 8 : MATLAB Function  TreatAsAtomicUnit=on
  choose ksi_est_err 9 : MATLAB Function  TreatAsAtomicUnit=on
  choose phi_1 : MATLAB Function  TreatAsAtomicUnit=on
  choose phi_2 : MATLAB Function  TreatAsAtomicUnit=on
  choose phi_3 : MATLAB Function  TreatAsAtomicUnit=on
  choose phi_4 : MATLAB Function  TreatAsAtomicUnit=on
  choose phi_5 : MATLAB Function  TreatAsAtomicUnit=on
  choose sigma_bar_v_1 : MATLAB Function  TreatAsAtomicUnit=on
  choose sigma_bar_v_2 : MATLAB Function  TreatAsAtomicUnit=on
  choose sigma_bar_v_3 : MATLAB Function  TreatAsAtomicUnit=on
  choose sigma_bar_v_4 : MATLAB Function  TreatAsAtomicUnit=on
  choose sigma_bar_v_5 : MATLAB Function  TreatAsAtomicUnit=on
  choose sigma_bar_v_hat_1 : MATLAB Function  TreatAsAtomicUnit=on
  choose sigma_bar_v_hat_2 : MATLAB Function  TreatAsAtomicUnit=on
  choose sigma_bar_v_hat_3 : MATLAB Function  TreatAsAtomicUnit=on
  choose sigma_bar_v_hat_4 : MATLAB Function  TreatAsAtomicUnit=on
  choose sigma_bar_v_hat_5 : MATLAB Function  TreatAsAtomicUnit=on
  choose sigma_bar_v_tilt_1 : MATLAB Function  TreatAsAtomicUnit=on
  choose sigma_bar_v_tilt_2 : MATLAB Function  TreatAsAtomicUnit=on
  choose sigma_bar_v_tilt_3 : MATLAB Function  TreatAsAtomicUnit=on
  choose sigma_bar_v_tilt_4 : MATLAB Function  TreatAsAtomicUnit=on
  choose sigma_bar_v_tilt_5 : MATLAB Function  TreatAsAtomicUnit=on
  choose ui agent 1 : MATLAB Function  TreatAsAtomicUnit=on
  choose ui agent 2 : MATLAB Function  TreatAsAtomicUnit=on
  choose ui agent 3 : MATLAB Function  TreatAsAtomicUnit=on
  choose ui agent 4 : MATLAB Function  TreatAsAtomicUnit=on
  choose ui agent 5 : MATLAB Function  TreatAsAtomicUnit=on
  combine Fi_S : MATLAB Function  TreatAsAtomicUnit=on
  combine Phi_bar_psi_e : MATLAB Function  TreatAsAtomicUnit=on
  combine Phi_psi_e : MATLAB Function  TreatAsAtomicUnit=on
  combine Qci Rci : MATLAB Function  TreatAsAtomicUnit=on
  combine Qci Rci1 : MATLAB Function  TreatAsAtomicUnit=on
  combine Qi Ri : MATLAB Function  TreatAsAtomicUnit=on
  combine S_bar : MATLAB Function  TreatAsAtomicUnit=on
  combine Si : MATLAB Function  TreatAsAtomicUnit=on
  combine Si_squ_beta_w_1 : MATLAB Function  TreatAsAtomicUnit=on
  combine Si_squ_beta_w_2 : MATLAB Function  TreatAsAtomicUnit=on
  combine V_Phi_Rei_squ_2p : MATLAB Function  TreatAsAtomicUnit=on
  combine V_Phi_Rei_squ_p_min_1 : MATLAB Function  TreatAsAtomicUnit=on
  combine V_Phi_Rei_squ_p_plus_1 : MATLAB Function  TreatAsAtomicUnit=on
  combine chi : MATLAB Function  TreatAsAtomicUnit=on
  combine d_sigma_bar_v_est : MATLAB Function  TreatAsAtomicUnit=on
  combine d_sigma_bar_v_est1 : MATLAB Function  TreatAsAtomicUnit=on
  combine dchi : MATLAB Function  TreatAsAtomicUnit=on
  combine dp_hat : MATLAB Function  TreatAsAtomicUnit=on
  combine dtheta_err_ksi : MATLAB Function  TreatAsAtomicUnit=on
  combine duihat d2uihat : MATLAB Function  TreatAsAtomicUnit=on
  combine dw_hat : MATLAB Function  TreatAsAtomicUnit=on
  combine dwi : MATLAB Function  TreatAsAtomicUnit=on
  combine follower desire velocity estimaters : MATLAB Function  TreatAsAtomicUnit=on
  combine follower eta ksi : MATLAB Function  TreatAsAtomicUnit=on
  combine formation control input : MATLAB Function  TreatAsAtomicUnit=on
  combine leader position estimaters : MATLAB Function  TreatAsAtomicUnit=on
  "combine lumped follower observation error " : MATLAB Function  TreatAsAtomicUnit=on
  combine lumped follower position observation error : MATLAB Function  TreatAsAtomicUnit=on
  combine lumped follower velocity observation error : MATLAB Function  TreatAsAtomicUnit=on
  combine norminal formation control input : MATLAB Function  TreatAsAtomicUnit=on
  combine rotational disturbance : MATLAB Function  TreatAsAtomicUnit=on
  combine sigma_bar_v_hat : MATLAB Function  TreatAsAtomicUnit=on
  combine sigma_bar_w_hat : MATLAB Function  TreatAsAtomicUnit=on
  combine sigma_v : MATLAB Function  TreatAsAtomicUnit=on
  combine sigma_w : MATLAB Function  TreatAsAtomicUnit=on
  combine tau : MATLAB Function  TreatAsAtomicUnit=on
  combine theta_Si_beta_w_1 : MATLAB Function  TreatAsAtomicUnit=on
  combine theta_Si_beta_w_2 : MATLAB Function  TreatAsAtomicUnit=on
  combine theta_err_ksi : MATLAB Function  TreatAsAtomicUnit=on
  combine theta_phi : MATLAB Function  TreatAsAtomicUnit=on
  combine theta_sigma_bar_v_tilt : MATLAB Function  TreatAsAtomicUnit=on
  combine theta_sigma_bar_w_tilt : MATLAB Function  TreatAsAtomicUnit=on
  combine translational disturbance : MATLAB Function  TreatAsAtomicUnit=on
  combine ui : MATLAB Function  TreatAsAtomicUnit=on
  combine wci dwci : MATLAB Function  TreatAsAtomicUnit=on
  combine wei Qei Rei : MATLAB Function  TreatAsAtomicUnit=on
  compare dp_1 and dp_hat_1 : Scope  NumInputPorts=3
  compare dp_2 and dp_hat_2 : Scope  NumInputPorts=3
  compare dp_3 and dp_hat_3 : Scope  NumInputPorts=3
  compare dp_4 and dp_hat_4 : Scope  NumInputPorts=3
  compare dp_5 and dp_hat_5 : Scope  NumInputPorts=3
  compare err_eta_1 and chi_1 : Scope  NumInputPorts=3
  compare err_eta_2 and chi_2 : Scope  NumInputPorts=3
  compare err_eta_3 and chi_3 : Scope  NumInputPorts=3
  compare err_eta_4 and chi_4 : Scope  NumInputPorts=3
  compare err_eta_5 and chi_5 : Scope  NumInputPorts=3
  compare sigma_bar_v_1 and sigma_bar_v_hat_1 : Scope  NumInputPorts=3
  compare sigma_bar_v_2 and sigma_bar_v_hat_2 : Scope  NumInputPorts=3
  compare sigma_bar_v_3 and sigma_bar_v_hat_3 : Scope  NumInputPorts=3
  compare sigma_bar_v_4 and sigma_bar_v_hat_4 : Scope  NumInputPorts=3
  compare sigma_bar_v_5 and sigma_bar_v_hat_5 : Scope  NumInputPorts=3
  control input generator agent 1 : MATLAB Function  TreatAsAtomicUnit=on
  control input generator agent 2 : MATLAB Function  TreatAsAtomicUnit=on
  control input generator agent 3 : MATLAB Function  TreatAsAtomicUnit=on
  control input generator agent 4 : MATLAB Function  TreatAsAtomicUnit=on
  control input generator agent 5 : MATLAB Function  TreatAsAtomicUnit=on
  d2_sigma_bar_v_est_{1..5} (5 alike) : Scope  NumInputPorts=3
  d2_sigma_bar_w_est_{1..5} (5 alike) : Scope  NumInputPorts=3
  d2_ui_hat_node_{1..5} (5 alike) : Scope  NumInputPorts=3
  d_sigma_bar_v_est_{1..5} (5 alike) : Scope  NumInputPorts=3
  d_sigma_bar_w_est_{1..5} (5 alike) : Scope  NumInputPorts=3
  d_ui_hat_node_{1..5} (5 alike) : Scope  NumInputPorts=3
  desire formation position and velocity : MATLAB Function  TreatAsAtomicUnit=on
  divide eta_est_err : MATLAB Function  TreatAsAtomicUnit=on
  divide ksi_est_err : MATLAB Function  TreatAsAtomicUnit=on
  dp_tilt_{1..5} (5 alike) : Scope  NumInputPorts=3
  dwci_node_{1..5} (5 alike) : Scope  NumInputPorts=3
  eta_0 : Scope  NumInputPorts=3
  eta_d_est_{1..5} (5 alike) : Scope  NumInputPorts=3
  eta_est_err_{1..5} (5 alike) : Scope  NumInputPorts=3
  eta_track_err_{1..5} (5 alike) : Scope  NumInputPorts=3
  fixed-time distributed follower desire position observer agent 1 : MATLAB Function  TreatAsAtomicUnit=on
  fixed-time distributed follower desire position observer agent 2 : MATLAB Function  TreatAsAtomicUnit=on
  fixed-time distributed follower desire position observer agent 3 : MATLAB Function  TreatAsAtomicUnit=on
  fixed-time distributed follower desire position observer agent 4 : MATLAB Function  TreatAsAtomicUnit=on
  fixed-time distributed follower desire position observer agent 5 : MATLAB Function  TreatAsAtomicUnit=on
  fixed-time distributed follower desire velocity observer agent 1 : MATLAB Function  TreatAsAtomicUnit=on
  fixed-time distributed follower desire velocity observer agent 2 : MATLAB Function  TreatAsAtomicUnit=on
  fixed-time distributed follower desire velocity observer agent 3 : MATLAB Function  TreatAsAtomicUnit=on
  fixed-time distributed follower desire velocity observer agent 4 : MATLAB Function  TreatAsAtomicUnit=on
  fixed-time distributed follower desire velocity observer agent 5 : MATLAB Function  TreatAsAtomicUnit=on
  follower etai Integrator agent 1 : Integrator  InitialCondition=etai_0(:,1)
  follower etai Integrator agent 2 : Integrator  InitialCondition=etai_0(:,2)
  follower etai Integrator agent 3 : Integrator  InitialCondition=etai_0(:,3)
  follower etai Integrator agent 4 : Integrator  InitialCondition=etai_0(:,4)
  follower etai Integrator agent 5 : Integrator  InitialCondition=etai_0(:,5)
  follower ksii Integrator agent 1 : Integrator  InitialCondition=ksii_0(:,1)
  follower ksii Integrator agent 2 : Integrator  InitialCondition=ksii_0(:,2)
  follower ksii Integrator agent 3 : Integrator  InitialCondition=ksii_0(:,3)
  follower ksii Integrator agent 4 : Integrator  InitialCondition=ksii_0(:,4)
  follower ksii Integrator agent 5 : Integrator  InitialCondition=ksii_0(:,5)
  follower tracking error agent 1 : MATLAB Function  TreatAsAtomicUnit=on
  follower tracking error agent 2 : MATLAB Function  TreatAsAtomicUnit=on
  follower tracking error agent 3 : MATLAB Function  TreatAsAtomicUnit=on
  follower tracking error agent 4 : MATLAB Function  TreatAsAtomicUnit=on
  follower tracking error agent 5 : MATLAB Function  TreatAsAtomicUnit=on
  generate angular rate disturbance agent 1 : MATLAB Function  TreatAsAtomicUnit=on
  generate angular rate disturbance agent 2 : MATLAB Function  TreatAsAtomicUnit=on
  generate angular rate disturbance agent 3 : MATLAB Function  TreatAsAtomicUnit=on
  generate angular rate disturbance agent 4 : MATLAB Function  TreatAsAtomicUnit=on
  generate angular rate disturbance agent 5 : MATLAB Function  TreatAsAtomicUnit=on
  generate translational disturbance agent 1 : MATLAB Function  TreatAsAtomicUnit=on
  generate translational disturbance agent 2 : MATLAB Function  TreatAsAtomicUnit=on
  generate translational disturbance agent 3 : MATLAB Function  TreatAsAtomicUnit=on
  generate translational disturbance agent 4 : MATLAB Function  TreatAsAtomicUnit=on
  generate translational disturbance agent 5 : MATLAB Function  TreatAsAtomicUnit=on
  ksi_0 : Scope  NumInputPorts=3
  ksi_d_est_{1..5} (5 alike) : Scope  NumInputPorts=3
  ksi_est_err_{1..5} (5 alike) : Scope  NumInputPorts=3
  ksi_track_err_{1..5} (5 alike) : Scope  NumInputPorts=3
  leader control input : MATLAB Function  TreatAsAtomicUnit=on
  leader eta0 Integrator : Integrator  ExternalReset=rising  InitialConditionSource=external  InitialCondition=vel0
  leader ksi0 Integrator : Integrator  InitialCondition=pos0
  phi_{1..5} (5 alike) : Scope  NumInputPorts=3
  position observe Integrator {1..5} (5 alike) : Integrator  InitialCondition=zeros(3,1)
  process velocity : MATLAB Function  TreatAsAtomicUnit=on
  set desire formation configuration : MATLAB Function  TreatAsAtomicUnit=on
  sigma_bar_v_hat Integrator {1..5} (5 alike) : Integrator  InitialCondition=zeros(3,1)
  sigma_bar_v_tilt_{1..5} (5 alike) : Scope  NumInputPorts=3
  sigma_bar_w_hat Integrator {1..5} (5 alike) : Integrator  InitialCondition=zeros(3,1)
  sigma_v Integrator {1..5} (5 alike) : Integrator  InitialCondition=zeros(3,1)
  trans to column1 : MATLAB Function  TreatAsAtomicUnit=on
  trans to column10 : MATLAB Function  TreatAsAtomicUnit=on
  trans to column100 : MATLAB Function  TreatAsAtomicUnit=on
  trans to column101 : MATLAB Function  TreatAsAtomicUnit=on
  trans to column102 : MATLAB Function  TreatAsAtomicUnit=on
  trans to column103 : MATLAB Function  TreatAsAtomicUnit=on
  trans to column104 : MATLAB Function  TreatAsAtomicUnit=on
  trans to column105 : MATLAB Function  TreatAsAtomicUnit=on
  trans to column106 : MATLAB Function  TreatAsAtomicUnit=on
  trans to column107 : MATLAB Function  TreatAsAtomicUnit=on
  trans to column108 : MATLAB Function  TreatAsAtomicUnit=on
  trans to column109 : MATLAB Function  TreatAsAtomicUnit=on
  trans to column11 : MATLAB Function  TreatAsAtomicUnit=on
  trans to column110 : MATLAB Function  TreatAsAtomicUnit=on
  trans to column111 : MATLAB Function  TreatAsAtomicUnit=on
  trans to column112 : MATLAB Function  TreatAsAtomicUnit=on
  trans to column113 : MATLAB Function  TreatAsAtomicUnit=on
  trans to column114 : MATLAB Function  TreatAsAtomicUnit=on
  trans to column115 : MATLAB Function  TreatAsAtomicUnit=on
  trans to column116 : MATLAB Function  TreatAsAtomicUnit=on
  trans to column117 : MATLAB Function  TreatAsAtomicUnit=on
  trans to column118 : MATLAB Function  TreatAsAtomicUnit=on
  trans to column119 : MATLAB Function  TreatAsAtomicUnit=on
  trans to column12 : MATLAB Function  TreatAsAtomicUnit=on
  trans to column120 : MATLAB Function  TreatAsAtomicUnit=on
  trans to column121 : MATLAB Function  TreatAsAtomicUnit=on
  trans to column122 : MATLAB Function  TreatAsAtomicUnit=on
  trans to column123 : MATLAB Function  TreatAsAtomicUnit=on
  trans to column124 : MATLAB Function  TreatAsAtomicUnit=on
  trans to column125 : MATLAB Function  TreatAsAtomicUnit=on
  trans to column13 : MATLAB Function  TreatAsAtomicUnit=on
  trans to column14 : MATLAB Function  TreatAsAtomicUnit=on
  trans to column15 : MATLAB Function  TreatAsAtomicUnit=on
  trans to column16 : MATLAB Function  TreatAsAtomicUnit=on
  trans to column17 : MATLAB Function  TreatAsAtomicUnit=on
  trans to column18 : MATLAB Function  TreatAsAtomicUnit=on
  trans to column19 : MATLAB Function  TreatAsAtomicUnit=on
  trans to column2 : MATLAB Function  TreatAsAtomicUnit=on
  trans to column20 : MATLAB Function  TreatAsAtomicUnit=on
  trans to column21 : MATLAB Function  TreatAsAtomicUnit=on
  trans to column22 : MATLAB Function  TreatAsAtomicUnit=on
  trans to column23 : MATLAB Function  TreatAsAtomicUnit=on
  trans to column24 : MATLAB Function  TreatAsAtomicUnit=on
  trans to column25 : MATLAB Function  TreatAsAtomicUnit=on
  trans to column26 : MATLAB Function  TreatAsAtomicUnit=on
  trans to column27 : MATLAB Function  TreatAsAtomicUnit=on
  trans to column28 : MATLAB Function  TreatAsAtomicUnit=on
  trans to column29 : MATLAB Function  TreatAsAtomicUnit=on
  trans to column3 : MATLAB Function  TreatAsAtomicUnit=on
  trans to column30 : MATLAB Function  TreatAsAtomicUnit=on
  trans to column31 : MATLAB Function  TreatAsAtomicUnit=on
  trans to column32 : MATLAB Function  TreatAsAtomicUnit=on
  trans to column33 : MATLAB Function  TreatAsAtomicUnit=on
  trans to column34 : MATLAB Function  TreatAsAtomicUnit=on
  trans to column35 : MATLAB Function  TreatAsAtomicUnit=on
  trans to column36 : MATLAB Function  TreatAsAtomicUnit=on
  trans to column37 : MATLAB Function  TreatAsAtomicUnit=on
  trans to column38 : MATLAB Function  TreatAsAtomicUnit=on
  trans to column39 : MATLAB Function  TreatAsAtomicUnit=on
  trans to column4 : MATLAB Function  TreatAsAtomicUnit=on
  trans to column40 : MATLAB Function  TreatAsAtomicUnit=on
  trans to column41 : MATLAB Function  TreatAsAtomicUnit=on
  trans to column42 : MATLAB Function  TreatAsAtomicUnit=on
  trans to column43 : MATLAB Function  TreatAsAtomicUnit=on
  trans to column44 : MATLAB Function  TreatAsAtomicUnit=on
  trans to column45 : MATLAB Function  TreatAsAtomicUnit=on
  trans to column46 : MATLAB Function  TreatAsAtomicUnit=on
  trans to column47 : MATLAB Function  TreatAsAtomicUnit=on
  trans to column48 : MATLAB Function  TreatAsAtomicUnit=on
  trans to column49 : MATLAB Function  TreatAsAtomicUnit=on
  trans to column5 : MATLAB Function  TreatAsAtomicUnit=on
  trans to column50 : MATLAB Function  TreatAsAtomicUnit=on
  trans to column51 : MATLAB Function  TreatAsAtomicUnit=on
  trans to column52 : MATLAB Function  TreatAsAtomicUnit=on
  trans to column53 : MATLAB Function  TreatAsAtomicUnit=on
  trans to column54 : MATLAB Function  TreatAsAtomicUnit=on
  trans to column55 : MATLAB Function  TreatAsAtomicUnit=on
  trans to column56 : MATLAB Function  TreatAsAtomicUnit=on
  trans to column57 : MATLAB Function  TreatAsAtomicUnit=on
  trans to column58 : MATLAB Function  TreatAsAtomicUnit=on
  trans to column59 : MATLAB Function  TreatAsAtomicUnit=on
  trans to column6 : MATLAB Function  TreatAsAtomicUnit=on
  trans to column60 : MATLAB Function  TreatAsAtomicUnit=on
  trans to column61 : MATLAB Function  TreatAsAtomicUnit=on
  trans to column62 : MATLAB Function  TreatAsAtomicUnit=on
  trans to column63 : MATLAB Function  TreatAsAtomicUnit=on
  trans to column64 : MATLAB Function  TreatAsAtomicUnit=on
  trans to column65 : MATLAB Function  TreatAsAtomicUnit=on
  trans to column66 : MATLAB Function  TreatAsAtomicUnit=on
  trans to column67 : MATLAB Function  TreatAsAtomicUnit=on
  trans to column68 : MATLAB Function  TreatAsAtomicUnit=on
  trans to column69 : MATLAB Function  TreatAsAtomicUnit=on
  trans to column7 : MATLAB Function  TreatAsAtomicUnit=on
  trans to column70 : MATLAB Function  TreatAsAtomicUnit=on
  trans to column71 : MATLAB Function  TreatAsAtomicUnit=on
  trans to column72 : MATLAB Function  TreatAsAtomicUnit=on
  trans to column73 : MATLAB Function  TreatAsAtomicUnit=on
  trans to column74 : MATLAB Function  TreatAsAtomicUnit=on
  trans to column75 : MATLAB Function  TreatAsAtomicUnit=on
  trans to column76 : MATLAB Function  TreatAsAtomicUnit=on
  trans to column77 : MATLAB Function  TreatAsAtomicUnit=on
  trans to column78 : MATLAB Function  TreatAsAtomicUnit=on
  trans to column79 : MATLAB Function  TreatAsAtomicUnit=on
  trans to column8 : MATLAB Function  TreatAsAtomicUnit=on
  trans to column80 : MATLAB Function  TreatAsAtomicUnit=on
  trans to column81 : MATLAB Function  TreatAsAtomicUnit=on
  trans to column82 : MATLAB Function  TreatAsAtomicUnit=on
  trans to column83 : MATLAB Function  TreatAsAtomicUnit=on
  trans to column84 : MATLAB Function  TreatAsAtomicUnit=on
  trans to column85 : MATLAB Function  TreatAsAtomicUnit=on
  trans to column86 : MATLAB Function  TreatAsAtomicUnit=on
  trans to column87 : MATLAB Function  TreatAsAtomicUnit=on
  trans to column88 : MATLAB Function  TreatAsAtomicUnit=on
  trans to column89 : MATLAB Function  TreatAsAtomicUnit=on
  trans to column9 : MATLAB Function  TreatAsAtomicUnit=on
  trans to column90 : MATLAB Function  TreatAsAtomicUnit=on
  trans to column91 : MATLAB Function  TreatAsAtomicUnit=on
  trans to column92 : MATLAB Function  TreatAsAtomicUnit=on
  trans to column93 : MATLAB Function  TreatAsAtomicUnit=on
  trans to column94 : MATLAB Function  TreatAsAtomicUnit=on
  trans to column95 : MATLAB Function  TreatAsAtomicUnit=on
  trans to column96 : MATLAB Function  TreatAsAtomicUnit=on
  trans to column97 : MATLAB Function  TreatAsAtomicUnit=on
  trans to column98 : MATLAB Function  TreatAsAtomicUnit=on
  trans to column99 : MATLAB Function  TreatAsAtomicUnit=on
  uav translational dynamics agent 1 : MATLAB Function  TreatAsAtomicUnit=on
  uav translational dynamics agent 2 : MATLAB Function  TreatAsAtomicUnit=on
  uav translational dynamics agent 3 : MATLAB Function  TreatAsAtomicUnit=on
  uav translational dynamics agent 4 : MATLAB Function  TreatAsAtomicUnit=on
  uav translational dynamics agent 5 : MATLAB Function  TreatAsAtomicUnit=on
  ui_tilt_node_{1..5} (5 alike) : Scope  NumInputPorts=3
  velocity observe Integrator {1..5} (5 alike) : Integrator  InitialCondition=zeros(3,1)
  virtual velocity tracking item agent 1 : MATLAB Function  TreatAsAtomicUnit=on
  virtual velocity tracking item agent 2 : MATLAB Function  TreatAsAtomicUnit=on
  virtual velocity tracking item agent 3 : MATLAB Function  TreatAsAtomicUnit=on
  virtual velocity tracking item agent 4 : MATLAB Function  TreatAsAtomicUnit=on
  virtual velocity tracking item agent 5 : MATLAB Function  TreatAsAtomicUnit=on
  wci_node_{1..5} (5 alike) : Scope  NumInputPorts=3
  wi dynam agent 1 : MATLAB Function  TreatAsAtomicUnit=on
  wi dynam agent 2 : MATLAB Function  TreatAsAtomicUnit=on
  wi dynam agent 3 : MATLAB Function  TreatAsAtomicUnit=on
  wi dynam agent 4 : MATLAB Function  TreatAsAtomicUnit=on
  wi dynam agent 5 : MATLAB Function  TreatAsAtomicUnit=on
  wires:
  [u0] -> To Workspace3/1
  [eta0] -> To Workspace4/1
  [ksi0] -> To Workspace5/1
  follower etai Integrator agent 1/1 -> [eta_1], follower ksii Integrator agent 1/1
  follower etai Integrator agent 2/1 -> [eta_2], follower ksii Integrator agent 2/1
  follower etai Integrator agent 3/1 -> [eta_3], follower ksii Integrator agent 3/1
  follower etai Integrator agent 4/1 -> [eta_4], follower ksii Integrator agent 4/1
  follower etai Integrator agent 5/1 -> [eta_5], follower ksii Integrator agent 5/1
  follower ksii Integrator agent 1/1 -> [ksi_1]
  follower ksii Integrator agent 2/1 -> [ksi_2]
  follower ksii Integrator agent 3/1 -> [ksi_3]
  follower ksii Integrator agent 4/1 -> [ksi_4]
  follower ksii Integrator agent 5/1 -> [ksi_5]
  [eta_1] -> combine formation control input/1(eta_1)
  [eta_2] -> combine formation control input/2(eta_2)
  [eta_3] -> combine formation control input/3(eta_3)
  [eta_4] -> combine formation control input/4(eta_4)
  [eta_5] -> combine formation control input/5(eta_5)
  [ksi_1] -> combine formation control input/6(ksi_1)
  [ksi_2] -> combine formation control input/7(ksi_2)
  [ksi_3] -> combine formation control input/8(ksi_3)
  [ksi_4] -> combine formation control input/9(ksi_4)
  [ksi_5] -> combine formation control input/10(ksi_5)
  [ksi_i_vec] -> follower tracking error agent 1/3(ksi_i_vec)
  [eta_i_vec] -> follower tracking error agent 1/4(eta_i_vec)
  [ksi0] -> follower tracking error agent 1/5(ksi0)
  [eta0] -> follower tracking error agent 1/6(eta0)
  follower tracking error agent 1/2(eta_track_err_1) -> Display13/1, Demux24/1, [eta_track_err_1]
  follower tracking error agent 1/1(ksi_track_err_1) -> Display12/1, Demux23/1, [ksi_track_err_1]
  [eta0] -> follower tracking error agent 2/6(eta0)
  [ksi0] -> follower tracking error agent 2/5(ksi0)
  [eta_i_vec] -> follower tracking error agent 2/4(eta_i_vec)
  follower tracking error agent 2/2(eta_track_err_2) -> Display15/1, Demux26/1, [eta_track_err_2]
  [ksi_i_vec] -> follower tracking error agent 2/3(ksi_i_vec)
  follower tracking error agent 2/1(ksi_track_err_2) -> Display14/1, Demux25/1, [ksi_track_err_2]
  follower tracking error agent 3/2(eta_track_err_3) -> Display17/1, Demux28/1, [eta_track_err_3]
  follower tracking error agent 3/1(ksi_track_err_3) -> Display16/1, Demux27/1, [ksi_track_err_3]
  [eta0] -> follower tracking error agent 3/6(eta0)
  [eta_i_vec] -> follower tracking error agent 3/4(eta_i_vec)
  [ksi_i_vec] -> follower tracking error agent 3/3(ksi_i_vec)
  [ksi0] -> follower tracking error agent 3/5(ksi0)
  [ksi_i_vec] -> follower tracking error agent 4/3(ksi_i_vec)
  [ksi0] -> follower tracking error agent 4/5(ksi0)
  [eta_i_vec] -> follower tracking error agent 4/4(eta_i_vec)
  [eta0] -> follower tracking error agent 4/6(eta0)
  follower tracking error agent 4/2(eta_track_err_4) -> Display19/1, Demux30/1, [eta_track_err_4]
  follower tracking error agent 4/1(ksi_track_err_4) -> Display18/1, Demux29/1, [ksi_track_err_4]
  follower tracking error agent 5/1(ksi_track_err_5) -> Display20/1, Demux31/1, [ksi_track_err_5]
  [ksi_i_vec] -> follower tracking error agent 5/3(ksi_i_vec)
  [eta0] -> follower tracking error agent 5/6(eta0)
  [ksi0] -> follower tracking error agent 5/5(ksi0)
  [eta_i_vec] -> follower tracking error agent 5/4(eta_i_vec)
  follower tracking error agent 5/2(eta_track_err_5) -> Display21/1, Demux32/1, [eta_track_err_5]
  [ksi_track_err_1] -> combine follower eta ksi/1(ksi_track_err_1)
  [ksi_track_err_2] -> combine follower eta ksi/2(ksi_track_err_2)
  [ksi_track_err_3] -> combine follower eta ksi/3(ksi_track_err_3)
  [ksi_track_err_4] -> combine follower eta ksi/4(ksi_track_err_4)
  [ksi_track_err_5] -> combine follower eta ksi/5(ksi_track_err_5)
  [eta_track_err_1] -> combine follower eta ksi/6(eta_track_err_1)
  [eta_track_err_2] -> combine follower eta ksi/7(eta_track_err_2)
  [eta_track_err_3] -> combine follower eta ksi/8(eta_track_err_3)
  [eta_track_err_4] -> combine follower eta ksi/9(eta_track_err_4)
  [eta_track_err_5] -> combine follower eta ksi/10(eta_track_err_5)
  combine follower eta ksi/1(ksi_track_err_vec) -> [ksi_track_err_vec]
  combine follower eta ksi/2(eta_track_err_vec) -> [eta_track_err_vec]
  [eta_i_vec] -> To Workspace7/1
  [ksi_i_vec] -> To Workspace8/1
  [ksi_track_err_vec] -> To Workspace9/1
  [eta_track_err_vec] -> To Workspace10/1
  Demux23/2 -> ksi_track_err_1/2
  Demux23/1 -> ksi_track_err_1/1
  Demux23/3 -> ksi_track_err_1/3
  Demux24/2 -> eta_track_err_1/2
  Demux24/1 -> eta_track_err_1/1
  Demux24/3 -> eta_track_err_1/3
  Demux25/2 -> ksi_track_err_2/2
  Demux25/1 -> ksi_track_err_2/1
  Demux25/3 -> ksi_track_err_2/3
  Demux26/1 -> eta_track_err_2/1
  Demux26/3 -> eta_track_err_2/3
  Demux26/2 -> eta_track_err_2/2
  Demux27/1 -> ksi_track_err_3/1
  Demux27/3 -> ksi_track_err_3/3
  Demux27/2 -> ksi_track_err_3/2
  Demux28/3 -> eta_track_err_3/3
  Demux28/2 -> eta_track_err_3/2
  Demux28/1 -> eta_track_err_3/1
  Demux29/3 -> ksi_track_err_4/3
  Demux29/2 -> ksi_track_err_4/2
  Demux29/1 -> ksi_track_err_4/1
  Demux30/3 -> eta_track_err_4/3
  Demux30/2 -> eta_track_err_4/2
  Demux30/1 -> eta_track_err_4/1
  Demux31/3 -> ksi_track_err_5/3
  Demux31/2 -> ksi_track_err_5/2
  Demux31/1 -> ksi_track_err_5/1
  Demux32/3 -> eta_track_err_5/3
  Demux32/2 -> eta_track_err_5/2
  Demux32/1 -> eta_track_err_5/1
  combine formation control input/1(eta_i_vec) -> Memory1/1
  Memory1/1 -> [eta_i_vec]
  combine formation control input/2(ksi_i_vec) -> Memory2/1
  Memory2/1 -> [ksi_i_vec]
  [ui_vec] -> To Workspace14/1
  [ui] -> uav translational dynamics agent 1/2(ui)
  [Ri] -> uav translational dynamics agent 1/1(Ri)
  uav translational dynamics agent 1/1(dvi) -> follower etai Integrator agent 1/1
  uav translational dynamics agent 2/1(dvi) -> follower etai Integrator agent 2/1
  [ui] -> uav translational dynamics agent 2/2(ui)
  [Ri] -> uav translational dynamics agent 2/1(Ri)
  [ui] -> uav translational dynamics agent 3/2(ui)
  [Ri] -> uav translational dynamics agent 3/1(Ri)
  uav translational dynamics agent 3/1(dvi) -> follower etai Integrator agent 3/1
  [ui] -> uav translational dynamics agent 4/2(ui)
  [Ri] -> uav translational dynamics agent 4/1(Ri)
  uav translational dynamics agent 4/1(dvi) -> follower etai Integrator agent 4/1
  [ui] -> uav translational dynamics agent 5/2(ui)
  [Ri] -> uav translational dynamics agent 5/1(Ri)
  uav translational dynamics agent 5/1(dvi) -> follower etai Integrator agent 5/1
  [ui] -> cal Rci from ui/2(ui)
  Constant191/1 -> cal Rci from ui/1(mi)
  cal Rei/1(Rei) -> [Rei]
  Constant51/1 -> cal Rei/1(Qei)
  [Rei] -> cal Ri/1(Rei)
  [Rci] -> cal Ri/2(Rci)
  cal Ri/1(Ri) -> [Ri]
  cal Rci from ui/1(Rci) -> [Rci]
  [tsim] -> generate translational disturbance agent 1/4(t)
  generate translational disturbance agent 1/1(dp_1) -> [dp_1]
  [dp_1] -> combine translational disturbance/1(dp_1)
  [dp_2] -> combine translational disturbance/2(dp_2)
  [dp_3] -> combine translational disturbance/3(dp_3)
  [dp_4] -> combine translational disturbance/4(dp_4)
  [dp_5] -> combine translational disturbance/5(dp_5)
  combine translational disturbance/1(dp_vec) -> [dp_vec]
  [dp_vec] -> uav translational dynamics agent 1/3(dp)
  [dp_vec] -> uav translational dynamics agent 2/3(dp)
  [dp_vec] -> uav translational dynamics agent 3/3(dp)
  [dp_vec] -> uav translational dynamics agent 4/3(dp)
  [dp_vec] -> uav translational dynamics agent 5/3(dp)
  Interpreted MATLAB Function1/1 -> trans to column1/1(x)
  Constant2/1 -> Mux30/2
  cal theta_err_ksi agent 1/1(theta_err_ksi_1_1) -> [theta_err_ksi_1_1]
  cal abs 2/1(y) -> Mux30/1
  choose ksi_est_err 1/1(y) -> cal abs 1/1(x)
  Constant3/1 -> Mux30/3
  [err_ksi_vec] -> choose ksi_est_err 2/1(x)
  [err_ksi_vec] -> choose ksi_est_err 1/1(x)
  cal abs 1/1(y) -> Mux36/1
  Interpreted MATLAB Function35/1 -> trans to column35/1(x)
  Constant1/1 -> Mux36/3
  Constant63/1 -> Mux36/2
  Mux36/1 -> Interpreted MATLAB Function35/1
  trans to column35/1(y) -> [err_ksi_squ_1_node_1], Display74/1
  cal theta_err_ksi agent 1/2(theta_err_ksi_2_1) -> [theta_err_ksi_2_1]
  trans to column1/1(y) -> [err_ksi_squ_2_node_1], Display1/1
  Mux30/1 -> Interpreted MATLAB Function1/1
  Constant16/1 -> cal theta_err_ksi agent 1/1(alfa_theta)
  [err_ksi_squ_2_node_1] -> cal theta_err_ksi agent 1/3(err_ksi_squ_2_node_1)
  choose ksi_est_err 2/1(y) -> cal abs 2/1(x)
  [err_ksi_squ_1_node_1] -> cal theta_err_ksi agent 1/2(err_ksi_squ_1_node_1)
  [err_ksi_vec] -> cal theta_err_ksi agent 1/4(err_ksi_vec)
  [err_ksi_vec] -> cal theta_err_ksi agent 2/4(err_ksi_vec)
  trans to column3/1(y) -> [err_ksi_squ_1_node_2], Display3/1
  Constant8/1 -> Mux2/2
  Constant4/1 -> Mux2/3
  Interpreted MATLAB Function3/1 -> trans to column3/1(x)
  [err_ksi_vec] -> choose ksi_est_err 3/1(x)
  [err_ksi_vec] -> choose ksi_est_err 4/1(x)
  choose ksi_est_err 3/1(y) -> cal abs 3/1(x)
  cal theta_err_ksi agent 2/1(theta_err_ksi_1_2) -> [theta_err_ksi_1_2]
  cal abs 4/1(y) -> Mux1/1
  Constant6/1 -> Mux1/2
  Interpreted MATLAB Function2/1 -> trans to column2/1(x)
  cal abs 3/1(y) -> Mux2/1
  choose ksi_est_err 4/1(y) -> cal abs 4/1(x)
  [err_ksi_squ_1_node_2] -> cal theta_err_ksi agent 2/2(err_ksi_squ_1_node_2)
  cal theta_err_ksi agent 2/2(theta_err_ksi_2_2) -> [theta_err_ksi_2_2]
  Mux1/1 -> Interpreted MATLAB Function2/1
  Constant5/1 -> cal theta_err_ksi agent 2/1(alfa_theta)
  trans to column2/1(y) -> [err_ksi_squ_2_node_2], Display2/1
  [err_ksi_squ_2_node_2] -> cal theta_err_ksi agent 2/3(err_ksi_squ_2_node_2)
  Constant7/1 -> Mux1/3
  Mux2/1 -> Interpreted MATLAB Function3/1
  [err_ksi_vec] -> choose ksi_est_err 6/1(x)
  Constant9/1 -> Mux4/3
  Constant13/1 -> Mux4/2
  trans to column5/1(y) -> [err_ksi_squ_1_node_3], Display5/1
  [err_ksi_vec] -> choose ksi_est_err 5/1(x)
  [err_ksi_vec] -> cal theta_err_ksi agent 3/4(err_ksi_vec)
  choose ksi_est_err 5/1(y) -> cal abs 5/1(x)
  [err_ksi_squ_2_node_3] -> cal theta_err_ksi agent 3/3(err_ksi_squ_2_node_3)
  trans to column4/1(y) -> [err_ksi_squ_2_node_3], Display4/1
  Mux4/1 -> Interpreted MATLAB Function5/1
  Constant10/1 -> cal theta_err_ksi agent 3/1(alfa_theta)
  Constant12/1 -> Mux3/3
  choose ksi_est_err 6/1(y) -> cal abs 6/1(x)
  Interpreted MATLAB Function5/1 -> trans to column5/1(x)
  [err_ksi_squ_1_node_3] -> cal theta_err_ksi agent 3/2(err_ksi_squ_1_node_3)
  cal theta_err_ksi agent 3/1(theta_err_ksi_1_3) -> [theta_err_ksi_1_3]
  cal abs 5/1(y) -> Mux4/1
  cal abs 6/1(y) -> Mux3/1
  Constant11/1 -> Mux3/2
  Interpreted MATLAB Function4/1 -> trans to column4/1(x)
  cal theta_err_ksi agent 3/2(theta_err_ksi_2_3) -> [theta_err_ksi_2_3]
  Mux3/1 -> Interpreted MATLAB Function4/1
  cal theta_err_ksi agent 4/2(theta_err_ksi_2_4) -> [theta_err_ksi_2_4]
  Constant15/1 -> Mux5/2
  Constant17/1 -> Mux5/3
  choose ksi_est_err 8/1(y) -> cal abs 8/1(x)
  cal abs 8/1(y) -> Mux5/1
  Constant14/1 -> cal theta_err_ksi agent 4/1(alfa_theta)
  cal theta_err_ksi agent 4/1(theta_err_ksi_1_4) -> [theta_err_ksi_1_4]
  [err_ksi_squ_1_node_4] -> cal theta_err_ksi agent 4/2(err_ksi_squ_1_node_4)
  cal abs 7/1(y) -> Mux6/1
  Interpreted MATLAB Function6/1 -> trans to column6/1(x)
  choose ksi_est_err 7/1(y) -> cal abs 7/1(x)
  [err_ksi_vec] -> cal theta_err_ksi agent 4/4(err_ksi_vec)
  trans to column6/1(y) -> [err_ksi_squ_2_node_4], Display7/1
  [err_ksi_squ_2_node_4] -> cal theta_err_ksi agent 4/3(err_ksi_squ_2_node_4)
  [err_ksi_vec] -> choose ksi_est_err 8/1(x)
  Mux5/1 -> Interpreted MATLAB Function6/1
  Constant18/1 -> Mux6/2
  trans to column7/1(y) -> [err_ksi_squ_1_node_4], Display8/1
  Interpreted MATLAB Function7/1 -> trans to column7/1(x)
  Mux6/1 -> Interpreted MATLAB Function7/1
  Constant19/1 -> Mux6/3
  [err_ksi_vec] -> choose ksi_est_err 7/1(x)
  Mux8/1 -> Interpreted MATLAB Function9/1
  Interpreted MATLAB Function9/1 -> trans to column9/1(x)
  [err_ksi_vec] -> choose ksi_est_err 9/1(x)
  Constant24/1 -> Mux8/3
  trans to column8/1(y) -> [err_ksi_squ_2_node_5], Display9/1
  Constant23/1 -> Mux8/2
  [err_ksi_squ_2_node_5] -> cal theta_err_ksi agent 5/3(err_ksi_squ_2_node_5)
  Mux7/1 -> Interpreted MATLAB Function8/1
  trans to column9/1(y) -> [err_ksi_squ_1_node_5], Display10/1
  choose ksi_est_err 9/1(y) -> cal abs 9/1(x)
  Interpreted MATLAB Function8/1 -> trans to column8/1(x)
  [err_ksi_vec] -> cal theta_err_ksi agent 5/4(err_ksi_vec)
  choose ksi_est_err 10/1(y) -> cal abs 10/1(x)
  [err_ksi_vec] -> choose ksi_est_err 10/1(x)
  [err_ksi_squ_1_node_5] -> cal theta_err_ksi agent 5/2(err_ksi_squ_1_node_5)
  cal abs 10/1(y) -> Mux7/1
  cal theta_err_ksi agent 5/1(theta_err_ksi_1_5) -> [theta_err_ksi_1_5]
  Constant22/1 -> Mux7/3
  Constant20/1 -> cal theta_err_ksi agent 5/1(alfa_theta)
  cal theta_err_ksi agent 5/2(theta_err_ksi_2_5) -> [theta_err_ksi_2_5]
  Constant21/1 -> Mux7/2
  cal abs 9/1(y) -> Mux8/1
  [theta_err_ksi_2_3] -> combine theta_err_ksi/8(theta_err_ksi_2_3)
  [theta_err_ksi_2_5] -> combine theta_err_ksi/10(theta_err_ksi_2_5)
  combine theta_err_ksi/2(theta_err_ksi_2_vec) -> [theta_err_ksi_2_vec]
  [theta_err_ksi_1_2] -> combine theta_err_ksi/2(theta_err_ksi_1_2)
  [theta_err_ksi_1_3] -> combine theta_err_ksi/3(theta_err_ksi_1_3)
  [theta_err_ksi_1_1] -> combine theta_err_ksi/1(theta_err_ksi_1_1)
  combine theta_err_ksi/1(theta_err_ksi_1_vec) -> [theta_err_ksi_1_vec]
  [theta_err_ksi_1_5] -> combine theta_err_ksi/5(theta_err_ksi_1_5)
  [theta_err_ksi_2_2] -> combine theta_err_ksi/7(theta_err_ksi_2_2)
  [theta_err_ksi_1_4] -> combine theta_err_ksi/4(theta_err_ksi_1_4)
  [theta_err_ksi_2_1] -> combine theta_err_ksi/6(theta_err_ksi_2_1)
  [theta_err_ksi_2_4] -> combine theta_err_ksi/9(theta_err_ksi_2_4)
  Constant26/1 -> virtual velocity tracking item agent 1/1(kai_chi_1)
  [theta_err_ksi_1_vec] -> virtual velocity tracking item agent 1/3(theta_err_ksi_1_vec)
  [theta_err_ksi_2_vec] -> virtual velocity tracking item agent 1/4(theta_err_ksi_2_vec)
  Constant25/1 -> virtual velocity tracking item agent 1/2(kai_chi_2)
  virtual velocity tracking item agent 1/1(chi_1) -> [chi_1]
  [theta_err_ksi_2_vec] -> virtual velocity tracking item agent 2/4(theta_err_ksi_2_vec)
  Constant28/1 -> virtual velocity tracking item agent 2/1(kai_chi_1)
  virtual velocity tracking item agent 2/1(chi_2) -> [chi_2]
  [theta_err_ksi_1_vec] -> virtual velocity tracking item agent 2/3(theta_err_ksi_1_vec)
  Constant27/1 -> virtual velocity tracking item agent 2/2(kai_chi_2)
  virtual velocity tracking item agent 3/1(chi_3) -> [chi_3]
  [theta_err_ksi_1_vec] -> virtual velocity tracking item agent 3/3(theta_err_ksi_1_vec)
  [theta_err_ksi_2_vec] -> virtual velocity tracking item agent 3/4(theta_err_ksi_2_vec)
  Constant29/1 -> virtual velocity tracking item agent 3/2(kai_chi_2)
  Constant30/1 -> virtual velocity tracking item agent 3/1(kai_chi_1)
  Constant32/1 -> virtual velocity tracking item agent 4/1(kai_chi_1)
  Constant31/1 -> virtual velocity tracking item agent 4/2(kai_chi_2)
  virtual velocity tracking item agent 4/1(chi_4) -> [chi_4]
  [theta_err_ksi_2_vec] -> virtual velocity tracking item agent 4/4(theta_err_ksi_2_vec)
  [theta_err_ksi_1_vec] -> virtual velocity tracking item agent 4/3(theta_err_ksi_1_vec)
  [theta_err_ksi_1_vec] -> virtual velocity tracking item agent 5/3(theta_err_ksi_1_vec)
  [theta_err_ksi_2_vec] -> virtual velocity tracking item agent 5/4(theta_err_ksi_2_vec)
  Constant34/1 -> virtual velocity tracking item agent 5/1(kai_chi_1)
  Constant33/1 -> virtual velocity tracking item agent 5/2(kai_chi_2)
  virtual velocity tracking item agent 5/1(chi_5) -> [chi_5]
  [chi_1] -> combine chi/1(chi_1)
  [chi_2] -> combine chi/2(chi_2)
  [chi_3] -> combine chi/3(chi_3)
  [chi_4] -> combine chi/4(chi_4)
  [chi_5] -> combine chi/5(chi_5)
  combine chi/1(chi_vec) -> [chi_vec]
  [err_eta_vec] -> cal virtual velocity control error phi/1(err_eta_vec)
  [chi_vec] -> cal virtual velocity control error phi/2(chi_vec)
  cal virtual velocity control error phi/1(phi_vec) -> [phi_vec]
  trans to column11/1(y) -> [d_err_ksi_squ_1_node_1], Display26/1
  Constant38/1 -> Mux10/2
  Constant35/1 -> Mux10/3
  Interpreted MATLAB Function11/1 -> trans to column11/1(x)
  [err_ksi_vec] -> choose ksi_est_err 11/1(x)
  [err_ksi_vec] -> choose ksi_est_err 12/1(x)
  choose ksi_est_err 11/1(y) -> cal abs 11/1(x)
  Constant36/1 -> Mux9/2
  cal abs 12/1(y) -> Mux9/1
  choose ksi_est_err 12/1(y) -> cal abs 12/1(x)
  Interpreted MATLAB Function10/1 -> trans to column10/1(x)
  cal abs 11/1(y) -> Mux10/1
  Mux9/1 -> Interpreted MATLAB Function10/1
  trans to column10/1(y) -> [d_err_ksi_squ_2_node_1], Display11/1
  Constant37/1 -> Mux9/3
  Mux10/1 -> Interpreted MATLAB Function11/1
  cal d_theta_err_ksi agent 1/1(d_theta_err_ksi_1_1) -> [d_theta_err_ksi_1_1]
  cal d_theta_err_ksi agent 1/2(d_theta_err_ksi_2_1) -> [d_theta_err_ksi_2_1]
  [err_ksi_vec] -> cal d_theta_err_ksi agent 1/8(err_ksi_vec)
  Constant39/1 -> cal d_theta_err_ksi agent 1/1(alfa_theta)
  [err_eta_vec] -> cal d_theta_err_ksi agent 1/9(err_eta_vec)
  [d_err_ksi_squ_2_node_1] -> cal d_theta_err_ksi agent 1/5(d_err_ksi_squ_2_node_1)
  [d_err_ksi_squ_1_node_1] -> cal d_theta_err_ksi agent 1/4(d_err_ksi_squ_1_node_1)
  Constant40/1 -> cal d_theta_err_ksi agent 1/2(beta1)
  Constant41/1 -> cal d_theta_err_ksi agent 1/3(beta2)
  [err_ksi_squ_2_node_1] -> cal d_theta_err_ksi agent 1/7(err_ksi_squ_2_node_1)
  [err_ksi_squ_1_node_1] -> cal d_theta_err_ksi agent 1/6(err_ksi_squ_1_node_1)
  [err_ksi_squ_1_node_2] -> cal d_theta_err_ksi agent 2/6(err_ksi_squ_1_node_2)
  Constant48/1 -> cal d_theta_err_ksi agent 2/3(beta2)
  [err_eta_vec] -> cal d_theta_err_ksi agent 2/9(err_eta_vec)
  Mux11/1 -> Interpreted MATLAB Function13/1
  [d_err_ksi_squ_1_node_2] -> cal d_theta_err_ksi agent 2/4(d_err_ksi_squ_1_node_2)
  Mux12/1 -> Interpreted MATLAB Function12/1
  Constant47/1 -> cal d_theta_err_ksi agent 2/2(beta1)
  Constant43/1 -> Mux12/2
  [err_ksi_vec] -> choose ksi_est_err 14/1(x)
  Interpreted MATLAB Function12/1 -> trans to column12/1(x)
  choose ksi_est_err 13/1(y) -> cal abs 13/1(x)
  cal abs 13/1(y) -> Mux11/1
  Constant44/1 -> Mux12/3
  choose ksi_est_err 14/1(y) -> cal abs 14/1(x)
  [d_err_ksi_squ_2_node_2] -> cal d_theta_err_ksi agent 2/5(d_err_ksi_squ_2_node_2)
  Constant45/1 -> Mux11/2
  Constant42/1 -> Mux11/3
  [err_ksi_vec] -> choose ksi_est_err 13/1(x)
  trans to column12/1(y) -> [d_err_ksi_squ_2_node_2], Display27/1
  Interpreted MATLAB Function13/1 -> trans to column13/1(x)
  cal abs 14/1(y) -> Mux12/1
  Constant46/1 -> cal d_theta_err_ksi agent 2/1(alfa_theta)
  cal d_theta_err_ksi agent 2/2(d_theta_err_ksi_2_2) -> [d_theta_err_ksi_2_2]
  cal d_theta_err_ksi agent 2/1(d_theta_err_ksi_1_2) -> [d_theta_err_ksi_1_2]
  [err_ksi_squ_2_node_2] -> cal d_theta_err_ksi agent 2/7(err_ksi_squ_2_node_2)
  [err_ksi_vec] -> cal d_theta_err_ksi agent 2/8(err_ksi_vec)
  trans to column13/1(y) -> [d_err_ksi_squ_1_node_2], Display28/1
  [err_ksi_squ_2_node_3] -> cal d_theta_err_ksi agent 3/7(err_ksi_squ_2_node_3)
  [err_ksi_vec] -> cal d_theta_err_ksi agent 3/8(err_ksi_vec)
  trans to column15/1(y) -> [d_err_ksi_squ_1_node_3], Display30/1
  cal abs 16/1(y) -> Mux14/1
  Constant54/1 -> cal d_theta_err_ksi agent 3/1(alfa_theta)
  cal d_theta_err_ksi agent 3/2(d_theta_err_ksi_2_3) -> [d_theta_err_ksi_2_3]
  Interpreted MATLAB Function15/1 -> trans to column15/1(x)
  cal d_theta_err_ksi agent 3/1(d_theta_err_ksi_1_3) -> [d_theta_err_ksi_1_3]
  Constant49/1 -> Mux13/3
  trans to column14/1(y) -> [d_err_ksi_squ_2_node_3], Display29/1
  [err_ksi_vec] -> choose ksi_est_err 15/1(x)
  Constant53/1 -> Mux13/2
  choose ksi_est_err 16/1(y) -> cal abs 16/1(x)
  choose ksi_est_err 15/1(y) -> cal abs 15/1(x)
  Constant52/1 -> Mux14/3
  cal abs 15/1(y) -> Mux13/1
  Interpreted MATLAB Function14/1 -> trans to column14/1(x)
  Constant55/1 -> cal d_theta_err_ksi agent 3/2(beta1)
  [d_err_ksi_squ_1_node_3] -> cal d_theta_err_ksi agent 3/4(d_err_ksi_squ_1_node_3)
  Constant56/1 -> cal d_theta_err_ksi agent 3/3(beta2)
  Mux13/1 -> Interpreted MATLAB Function15/1
  [d_err_ksi_squ_2_node_3] -> cal d_theta_err_ksi agent 3/5(d_err_ksi_squ_2_node_3)
  Constant50/1 -> Mux14/2
  [err_eta_vec] -> cal d_theta_err_ksi agent 3/9(err_eta_vec)
  Mux14/1 -> Interpreted MATLAB Function14/1
  [err_ksi_vec] -> choose ksi_est_err 16/1(x)
  [err_ksi_squ_1_node_3] -> cal d_theta_err_ksi agent 3/6(err_ksi_squ_1_node_3)
  [err_ksi_vec] -> choose ksi_est_err 18/1(x)
  Mux15/1 -> Interpreted MATLAB Function17/1
  Interpreted MATLAB Function16/1 -> trans to column16/1(x)
  [err_eta_vec] -> cal d_theta_err_ksi agent 4/9(err_eta_vec)
  Mux16/1 -> Interpreted MATLAB Function16/1
  Constant58/1 -> Mux16/2
  Constant62/1 -> cal d_theta_err_ksi agent 4/2(beta1)
  [d_err_ksi_squ_1_node_4] -> cal d_theta_err_ksi agent 4/4(d_err_ksi_squ_1_node_4)
  [d_err_ksi_squ_2_node_4] -> cal d_theta_err_ksi agent 4/5(d_err_ksi_squ_2_node_4)
  cal abs 17/1(y) -> Mux15/1
  [err_ksi_squ_1_node_4] -> cal d_theta_err_ksi agent 4/6(err_ksi_squ_1_node_4)
  trans to column16/1(y) -> [d_err_ksi_squ_2_node_4], Display31/1
  Constant59/1 -> Mux16/3
  Constant74/1 -> cal d_theta_err_ksi agent 4/3(beta2)
  choose ksi_est_err 17/1(y) -> cal abs 17/1(x)
  choose ksi_est_err 18/1(y) -> cal abs 18/1(x)
  Constant60/1 -> Mux15/2
  [err_ksi_vec] -> choose ksi_est_err 17/1(x)
  cal abs 18/1(y) -> Mux16/1
  Interpreted MATLAB Function17/1 -> trans to column17/1(x)
  Constant57/1 -> Mux15/3
  trans to column17/1(y) -> [d_err_ksi_squ_1_node_4], Display32/1
  cal d_theta_err_ksi agent 4/1(d_theta_err_ksi_1_4) -> [d_theta_err_ksi_1_4]
  [err_ksi_vec] -> cal d_theta_err_ksi agent 4/8(err_ksi_vec)
  Constant61/1 -> cal d_theta_err_ksi agent 4/1(alfa_theta)
  [err_ksi_squ_2_node_4] -> cal d_theta_err_ksi agent 4/7(err_ksi_squ_2_node_4)
  cal d_theta_err_ksi agent 4/2(d_theta_err_ksi_2_4) -> [d_theta_err_ksi_2_4]
  [d_err_ksi_squ_2_node_5] -> cal d_theta_err_ksi agent 5/5(d_err_ksi_squ_2_node_5)
  Constant80/1 -> cal d_theta_err_ksi agent 5/2(beta1)
  Constant76/1 -> Mux18/2
  [d_err_ksi_squ_1_node_5] -> cal d_theta_err_ksi agent 5/4(d_err_ksi_squ_1_node_5)
  Mux18/1 -> Interpreted MATLAB Function18/1
  Interpreted MATLAB Function18/1 -> trans to column18/1(x)
  [err_eta_vec] -> cal d_theta_err_ksi agent 5/9(err_eta_vec)
  cal d_theta_err_ksi agent 5/2(d_theta_err_ksi_2_5) -> [d_theta_err_ksi_2_5]
  [err_ksi_squ_2_node_5] -> cal d_theta_err_ksi agent 5/7(err_ksi_squ_2_node_5)
  [err_ksi_vec] -> choose ksi_est_err 20/1(x)
  [err_ksi_vec] -> cal d_theta_err_ksi agent 5/8(err_ksi_vec)
  trans to column19/1(y) -> [d_err_ksi_squ_1_node_5], Display34/1
  Constant79/1 -> cal d_theta_err_ksi agent 5/1(alfa_theta)
  Constant75/1 -> Mux17/3
  Interpreted MATLAB Function19/1 -> trans to column19/1(x)
  [err_ksi_vec] -> choose ksi_est_err 19/1(x)
  cal abs 20/1(y) -> Mux18/1
  Constant78/1 -> Mux17/2
  Constant77/1 -> Mux18/3
  choose ksi_est_err 20/1(y) -> cal abs 20/1(x)
  [err_ksi_squ_1_node_5] -> cal d_theta_err_ksi agent 5/6(err_ksi_squ_1_node_5)
  cal d_theta_err_ksi agent 5/1(d_theta_err_ksi_1_5) -> [d_theta_err_ksi_1_5]
  choose ksi_est_err 19/1(y) -> cal abs 19/1(x)
  Constant81/1 -> cal d_theta_err_ksi agent 5/3(beta2)
  Mux17/1 -> Interpreted MATLAB Function19/1
  trans to column18/1(y) -> [d_err_ksi_squ_2_node_5], Display33/1
  cal abs 19/1(y) -> Mux17/1
  [d_theta_err_ksi_2_vec] -> cal dchi agent 1/4(d_theta_err_ksi_2_vec)
  Constant83/1 -> cal dchi agent 1/1(kai_chi_1)
  cal dchi agent 1/1(d_chi_1) -> [d_chi_1]
  [d_theta_err_ksi_1_vec] -> cal dchi agent 1/3(d_theta_err_ksi_1_vec)
  Constant82/1 -> cal dchi agent 1/2(kai_chi_2)
  combine dtheta_err_ksi/1(d_theta_err_ksi_1_vec) -> [d_theta_err_ksi_1_vec]
  [d_theta_err_ksi_2_1] -> combine dtheta_err_ksi/6(d_theta_err_ksi_2_1)
  [d_theta_err_ksi_1_4] -> combine dtheta_err_ksi/4(d_theta_err_ksi_1_4)
  [d_theta_err_ksi_2_2] -> combine dtheta_err_ksi/7(d_theta_err_ksi_2_2)
  [d_theta_err_ksi_1_2] -> combine dtheta_err_ksi/2(d_theta_err_ksi_1_2)
  [d_theta_err_ksi_2_5] -> combine dtheta_err_ksi/10(d_theta_err_ksi_2_5)
  [d_theta_err_ksi_2_4] -> combine dtheta_err_ksi/9(d_theta_err_ksi_2_4)
  combine dtheta_err_ksi/2(d_theta_err_ksi_2_vec) -> [d_theta_err_ksi_2_vec]
  [d_theta_err_ksi_1_1] -> combine dtheta_err_ksi/1(d_theta_err_ksi_1_1)
  [d_theta_err_ksi_2_3] -> combine dtheta_err_ksi/8(d_theta_err_ksi_2_3)
  [d_theta_err_ksi_1_5] -> combine dtheta_err_ksi/5(d_theta_err_ksi_1_5)
  [d_theta_err_ksi_1_3] -> combine dtheta_err_ksi/3(d_theta_err_ksi_1_3)
  cal dchi agent 2/1(d_chi_2) -> [d_chi_2]
  [d_theta_err_ksi_1_vec] -> cal dchi agent 2/3(d_theta_err_ksi_1_vec)
  Constant85/1 -> cal dchi agent 2/1(kai_chi_1)
  Constant84/1 -> cal dchi agent 2/2(kai_chi_2)
  [d_theta_err_ksi_2_vec] -> cal dchi agent 2/4(d_theta_err_ksi_2_vec)
  [d_theta_err_ksi_2_vec] -> cal dchi agent 3/4(d_theta_err_ksi_2_vec)
  Constant87/1 -> cal dchi agent 3/1(kai_chi_1)
  [d_theta_err_ksi_1_vec] -> cal dchi agent 3/3(d_theta_err_ksi_1_vec)
  cal dchi agent 3/1(d_chi_3) -> [d_chi_3]
  Constant86/1 -> cal dchi agent 3/2(kai_chi_2)
  Constant88/1 -> cal dchi agent 4/2(kai_chi_2)
  Constant89/1 -> cal dchi agent 4/1(kai_chi_1)
  cal dchi agent 4/1(d_chi_4) -> [d_chi_4]
  [d_theta_err_ksi_1_vec] -> cal dchi agent 4/3(d_theta_err_ksi_1_vec)
  [d_theta_err_ksi_2_vec] -> cal dchi agent 4/4(d_theta_err_ksi_2_vec)
  Constant91/1 -> cal dchi agent 5/1(kai_chi_1)
  [d_theta_err_ksi_1_vec] -> cal dchi agent 5/3(d_theta_err_ksi_1_vec)
  cal dchi agent 5/1(d_chi_5) -> [d_chi_5]
  Constant90/1 -> cal dchi agent 5/2(kai_chi_2)
  [d_theta_err_ksi_2_vec] -> cal dchi agent 5/4(d_theta_err_ksi_2_vec)
  [d_chi_4] -> combine dchi/4(d_chi_4)
  combine dchi/1(d_chi_vec) -> [d_chi_vec]
  [d_chi_5] -> combine dchi/5(d_chi_5)
  [d_chi_2] -> combine dchi/2(d_chi_2)
  [d_chi_1] -> combine dchi/1(d_chi_1)
  [d_chi_3] -> combine dchi/3(d_chi_3)
  [Ri] -> cal virtual control sigma_v agent 1/2(Ri)
  [ui] -> cal virtual control sigma_v agent 1/3(ui_vec)
  Constant92/1 -> cal virtual control sigma_v agent 1/1(c3v)
  [sigma_bar_v_vec] -> cal virtual control sigma_v agent 1/4(sigma_bar_v_vec)
  cal virtual control sigma_v agent 1/1(d_sigma_v_1) -> sigma_v Integrator 1/1
  sigma_v Integrator 1/1 -> [sigma_v_1]
  [sigma_bar_v_vec] -> cal virtual control sigma_v agent 2/4(sigma_bar_v_vec)
  sigma_v Integrator 2/1 -> [sigma_v_2]
  Constant93/1 -> cal virtual control sigma_v agent 2/1(c3v)
  [Ri] -> cal virtual control sigma_v agent 2/2(Ri)
  cal virtual control sigma_v agent 2/1(d_sigma_v_2) -> sigma_v Integrator 2/1
  [ui] -> cal virtual control sigma_v agent 2/3(ui_vec)
  Constant94/1 -> cal virtual control sigma_v agent 3/1(c3v)
  cal virtual control sigma_v agent 3/1(d_sigma_v_3) -> sigma_v Integrator 3/1
  [ui] -> cal virtual control sigma_v agent 3/3(ui_vec)
  [Ri] -> cal virtual control sigma_v agent 3/2(Ri)
  [sigma_bar_v_vec] -> cal virtual control sigma_v agent 3/4(sigma_bar_v_vec)
  sigma_v Integrator 3/1 -> [sigma_v_3]
  sigma_v Integrator 4/1 -> [sigma_v_4]
  [Ri] -> cal virtual control sigma_v agent 4/2(Ri)
  [sigma_bar_v_vec] -> cal virtual control sigma_v agent 4/4(sigma_bar_v_vec)
  [ui] -> cal virtual control sigma_v agent 4/3(ui_vec)
  cal virtual control sigma_v agent 4/1(d_sigma_v_4) -> sigma_v Integrator 4/1
  Constant95/1 -> cal virtual control sigma_v agent 4/1(c3v)
  Constant96/1 -> cal virtual control sigma_v agent 5/1(c3v)
  [sigma_bar_v_vec] -> cal virtual control sigma_v agent 5/4(sigma_bar_v_vec)
  [Ri] -> cal virtual control sigma_v agent 5/2(Ri)
  [ui] -> cal virtual control sigma_v agent 5/3(ui_vec)
  sigma_v Integrator 5/1 -> [sigma_v_5]
  cal virtual control sigma_v agent 5/1(d_sigma_v_5) -> sigma_v Integrator 5/1
  combine sigma_v/1(sigma_v_vec) -> [sigma_v_vec]
  [sigma_v_4] -> combine sigma_v/4(sigma_v_4)
  [sigma_v_3] -> combine sigma_v/3(sigma_v_3)
  [sigma_v_1] -> combine sigma_v/1(sigma_v_1)
  [sigma_v_5] -> combine sigma_v/5(sigma_v_5)
  [sigma_v_2] -> combine sigma_v/2(sigma_v_2)
  [eta_i_vec] -> cal combine sigma_bar_v/1(eta_i_vec)
  [sigma_v_vec] -> cal combine sigma_bar_v/2(sigma_v_vec)
  cal combine sigma_bar_v/1(sigma_bar_v_vec) -> [sigma_bar_v_vec]
  Demux12/3 -> d2_sigma_bar_v_est_1/3
  Demux12/2 -> d2_sigma_bar_v_est_1/2
  Demux8/3 -> d_sigma_bar_v_est_1/3
  Demux12/1 -> d2_sigma_bar_v_est_1/1
  Demux8/1 -> d_sigma_bar_v_est_1/1
  Demux8/2 -> d_sigma_bar_v_est_1/2
  cal differentiator d_sigma_bar_v_hat agent 1/1(Out1) -> Display35/1, [sigma_bar_v_est_1]
  cal differentiator d_sigma_bar_v_hat agent 1/2(Out2) -> Demux8/1, [d_sigma_bar_v_est_1], Display36/1
  cal differentiator d_sigma_bar_v_hat agent 1/3(Out3) -> Demux12/1, [d2_sigma_bar_v_est_1], Display37/1
  [sigma_bar_v_vec] -> cal differentiator d_sigma_bar_v_hat agent 1/1(x)
  cal differentiator d_sigma_bar_v_hat agent 2/1(Out1) -> Display38/1, [sigma_bar_v_est_2]
  [sigma_bar_v_vec] -> cal differentiator d_sigma_bar_v_hat agent 2/1(x)
  cal differentiator d_sigma_bar_v_hat agent 2/2(Out2) -> Demux3/1, [d_sigma_bar_v_est_2], Display39/1
  cal differentiator d_sigma_bar_v_hat agent 2/3(Out3) -> Demux2/1, [d2_sigma_bar_v_est_2], Display40/1
  Demux2/2 -> d2_sigma_bar_v_est_2/2
  Demux2/3 -> d2_sigma_bar_v_est_2/3
  Demux3/2 -> d_sigma_bar_v_est_2/2
  Demux2/1 -> d2_sigma_bar_v_est_2/1
  Demux3/1 -> d_sigma_bar_v_est_2/1
  Demux3/3 -> d_sigma_bar_v_est_2/3
  Demux5/1 -> d_sigma_bar_v_est_3/1
  Demux5/3 -> d_sigma_bar_v_est_3/3
  Demux4/2 -> d2_sigma_bar_v_est_3/2
  Demux4/3 -> d2_sigma_bar_v_est_3/3
  Demux5/2 -> d_sigma_bar_v_est_3/2
  Demux4/1 -> d2_sigma_bar_v_est_3/1
  cal differentiator d_sigma_bar_v_hat agent 3/3(Out3) -> Demux4/1, [d2_sigma_bar_v_est_3], Display43/1
  cal differentiator d_sigma_bar_v_hat agent 3/2(Out2) -> Demux5/1, [d_sigma_bar_v_est_3], Display42/1
  cal differentiator d_sigma_bar_v_hat agent 3/1(Out1) -> Display41/1, [sigma_bar_v_est_3]
  [sigma_bar_v_vec] -> cal differentiator d_sigma_bar_v_hat agent 3/1(x)
  cal differentiator d_sigma_bar_v_hat agent 4/3(Out3) -> Demux6/1, [d2_sigma_bar_v_est_4], Display46/1
  Demux6/1 -> d2_sigma_bar_v_est_4/1
  Demux6/3 -> d2_sigma_bar_v_est_4/3
  Demux7/2 -> d_sigma_bar_v_est_4/2
  Demux6/2 -> d2_sigma_bar_v_est_4/2
  Demux7/3 -> d_sigma_bar_v_est_4/3
  Demux7/1 -> d_sigma_bar_v_est_4/1
  cal differentiator d_sigma_bar_v_hat agent 4/1(Out1) -> Display44/1, [sigma_bar_v_est_4]
  cal differentiator d_sigma_bar_v_hat agent 4/2(Out2) -> Demux7/1, [d_sigma_bar_v_est_4], Display45/1
  [sigma_bar_v_vec] -> cal differentiator d_sigma_bar_v_hat agent 4/1(x)
  cal differentiator d_sigma_bar_v_hat agent 5/1(Out1) -> Display47/1, [sigma_bar_v_est_5]
  cal differentiator d_sigma_bar_v_hat agent 5/2(Out2) -> Demux10/1, [d_sigma_bar_v_est_5], Display48/1
  [sigma_bar_v_vec] -> cal differentiator d_sigma_bar_v_hat agent 5/1(x)
  Demux10/3 -> d_sigma_bar_v_est_5/3
  Demux9/2 -> d2_sigma_bar_v_est_5/2
  Demux10/2 -> d_sigma_bar_v_est_5/2
  Demux9/1 -> d2_sigma_bar_v_est_5/1
  cal differentiator d_sigma_bar_v_hat agent 5/3(Out3) -> Demux9/1, [d2_sigma_bar_v_est_5], Display49/1
  Demux10/1 -> d_sigma_bar_v_est_5/1
  Demux9/3 -> d2_sigma_bar_v_est_5/3
  [d_sigma_bar_v_est_5] -> combine d_sigma_bar_v_est/5(d_sigma_bar_v_est_5)
  [d_sigma_bar_v_est_2] -> combine d_sigma_bar_v_est/2(d_sigma_bar_v_est_2)
  [d_sigma_bar_v_est_1] -> combine d_sigma_bar_v_est/1(d_sigma_bar_v_est_1)
  [d_sigma_bar_v_est_4] -> combine d_sigma_bar_v_est/4(d_sigma_bar_v_est_4)
  [d_sigma_bar_v_est_3] -> combine d_sigma_bar_v_est/3(d_sigma_bar_v_est_3)
  combine d_sigma_bar_v_est/1(d_sigma_bar_v_vec) -> [d_sigma_bar_v_vec]
  trans to column21/1(y) -> [sigma_bar_v_tilt_squ_1_1], Display51/1
  Constant100/1 -> Mux20/2
  Constant97/1 -> Mux20/3
  Interpreted MATLAB Function21/1 -> trans to column21/1(x)
  [sigma_bar_v_tilt_vec] -> choose ksi_est_err 21/1(x)
  choose ksi_est_err 21/1(y) -> cal abs 21/1(x)
  Constant98/1 -> Mux19/2
  cal abs 22/1(y) -> Mux19/1
  choose ksi_est_err 22/1(y) -> cal abs 22/1(x)
  Interpreted MATLAB Function20/1 -> trans to column20/1(x)
  cal abs 21/1(y) -> Mux20/1
  Mux19/1 -> Interpreted MATLAB Function20/1
  trans to column20/1(y) -> [sigma_bar_v_tilt_squ_2_1], Display50/1
  Constant99/1 -> Mux19/3
  Mux20/1 -> Interpreted MATLAB Function21/1
  [sigma_bar_v_tilt_vec] -> choose ksi_est_err 22/1(x)
  cal theta_sigma_bar_v_tilt agent 1/1(theta_sigma_bar_v_tilt_1_1) -> [theta_sigma_bar_v_tilt_1_1]
  [sigma_bar_v_tilt_squ_1_1] -> cal theta_sigma_bar_v_tilt agent 1/2(sigma_bar_v_tilt_squ_1_1)
  cal theta_sigma_bar_v_tilt agent 1/2(theta_sigma_bar_v_tilt_2_1) -> [theta_sigma_bar_v_tilt_2_1]
  [sigma_bar_v_tilt_vec] -> cal theta_sigma_bar_v_tilt agent 1/4(sigma_bar_v_tilt_vec)
  [sigma_bar_v_tilt_squ_2_1] -> cal theta_sigma_bar_v_tilt agent 1/3(sigma_bar_v_tilt_squ_2_1)
  Constant101/1 -> cal theta_sigma_bar_v_tilt agent 1/1(alfa_theta)
  Constant103/1 -> cal theta_sigma_bar_v_tilt agent 2/1(alfa_theta)
  [sigma_bar_v_tilt_vec] -> cal theta_sigma_bar_v_tilt agent 2/4(sigma_bar_v_tilt_vec)
  [sigma_bar_v_tilt_squ_1_2] -> cal theta_sigma_bar_v_tilt agent 2/2(sigma_bar_v_tilt_squ_1_2)
  trans to column23/1(y) -> [sigma_bar_v_tilt_squ_1_2], Display53/1
  Interpreted MATLAB Function23/1 -> trans to column23/1(x)
  Mux22/1 -> Interpreted MATLAB Function23/1
  Constant106/1 -> Mux21/3
  cal theta_sigma_bar_v_tilt agent 2/1(theta_sigma_bar_v_tilt_1_2) -> [theta_sigma_bar_v_tilt_1_2]
  Constant102/1 -> Mux22/2
  trans to column22/1(y) -> [sigma_bar_v_tilt_squ_2_2], Display52/1
  Interpreted MATLAB Function22/1 -> trans to column22/1(x)
  cal abs 23/1(y) -> Mux22/1
  Constant104/1 -> Mux22/3
  Mux21/1 -> Interpreted MATLAB Function22/1
  choose ksi_est_err 24/1(y) -> cal abs 24/1(x)
  cal abs 24/1(y) -> Mux21/1
  choose ksi_est_err 23/1(y) -> cal abs 23/1(x)
  [sigma_bar_v_tilt_vec] -> choose ksi_est_err 24/1(x)
  [sigma_bar_v_tilt_squ_2_2] -> cal theta_sigma_bar_v_tilt agent 2/3(sigma_bar_v_tilt_squ_2_2)
  Constant105/1 -> Mux21/2
  [sigma_bar_v_tilt_vec] -> choose ksi_est_err 23/1(x)
  cal theta_sigma_bar_v_tilt agent 2/2(theta_sigma_bar_v_tilt_2_2) -> [theta_sigma_bar_v_tilt_2_2]
  [sigma_bar_v_tilt_vec] -> choose ksi_est_err 25/1(x)
  cal theta_sigma_bar_v_tilt agent 3/2(theta_sigma_bar_v_tilt_2_3) -> [theta_sigma_bar_v_tilt_2_3]
  Constant110/1 -> Mux23/2
  [sigma_bar_v_tilt_squ_2_3] -> cal theta_sigma_bar_v_tilt agent 3/3(sigma_bar_v_tilt_squ_2_3)
  [sigma_bar_v_tilt_vec] -> choose ksi_est_err 26/1(x)
  choose ksi_est_err 25/1(y) -> cal abs 25/1(x)
  Mux23/1 -> Interpreted MATLAB Function24/1
  choose ksi_est_err 26/1(y) -> cal abs 26/1(x)
  Constant109/1 -> Mux24/3
  cal abs 25/1(y) -> Mux24/1
  Interpreted MATLAB Function24/1 -> trans to column24/1(x)
  Constant107/1 -> Mux24/2
  Mux24/1 -> Interpreted MATLAB Function25/1
  cal theta_sigma_bar_v_tilt agent 3/1(theta_sigma_bar_v_tilt_1_3) -> [theta_sigma_bar_v_tilt_1_3]
  Constant111/1 -> Mux23/3
  Constant108/1 -> cal theta_sigma_bar_v_tilt agent 3/1(alfa_theta)
  trans to column24/1(y) -> [sigma_bar_v_tilt_squ_2_3], Display54/1
  [sigma_bar_v_tilt_squ_1_3] -> cal theta_sigma_bar_v_tilt agent 3/2(sigma_bar_v_tilt_squ_1_3)
  trans to column25/1(y) -> [sigma_bar_v_tilt_squ_1_3], Display55/1
  Interpreted MATLAB Function25/1 -> trans to column25/1(x)
  [sigma_bar_v_tilt_vec] -> cal theta_sigma_bar_v_tilt agent 3/4(sigma_bar_v_tilt_vec)
  cal abs 26/1(y) -> Mux23/1
  cal abs 28/1(y) -> Mux25/1
  trans to column27/1(y) -> [sigma_bar_v_tilt_squ_1_4], Display57/1
  Interpreted MATLAB Function27/1 -> trans to column27/1(x)
  Constant113/1 -> cal theta_sigma_bar_v_tilt agent 4/1(alfa_theta)
  [sigma_bar_v_tilt_squ_1_4] -> cal theta_sigma_bar_v_tilt agent 4/2(sigma_bar_v_tilt_squ_1_4)
  Constant116/1 -> Mux25/3
  trans to column26/1(y) -> [sigma_bar_v_tilt_squ_2_4], Display56/1
  Constant112/1 -> Mux26/2
  Mux26/1 -> Interpreted MATLAB Function27/1
  [sigma_bar_v_tilt_vec] -> cal theta_sigma_bar_v_tilt agent 4/4(sigma_bar_v_tilt_vec)
  Constant114/1 -> Mux26/3
  cal abs 27/1(y) -> Mux26/1
  cal theta_sigma_bar_v_tilt agent 4/1(theta_sigma_bar_v_tilt_1_4) -> [theta_sigma_bar_v_tilt_1_4]
  Constant115/1 -> Mux25/2
  choose ksi_est_err 27/1(y) -> cal abs 27/1(x)
  choose ksi_est_err 28/1(y) -> cal abs 28/1(x)
  Interpreted MATLAB Function26/1 -> trans to column26/1(x)
  cal theta_sigma_bar_v_tilt agent 4/2(theta_sigma_bar_v_tilt_2_4) -> [theta_sigma_bar_v_tilt_2_4]
  [sigma_bar_v_tilt_vec] -> choose ksi_est_err 28/1(x)
  [sigma_bar_v_tilt_squ_2_4] -> cal theta_sigma_bar_v_tilt agent 4/3(sigma_bar_v_tilt_squ_2_4)
  [sigma_bar_v_tilt_vec] -> choose ksi_est_err 27/1(x)
  Mux25/1 -> Interpreted MATLAB Function26/1
  [sigma_bar_v_tilt_squ_2_5] -> cal theta_sigma_bar_v_tilt agent 5/3(sigma_bar_v_tilt_squ_2_5)
  choose ksi_est_err 29/1(y) -> cal abs 29/1(x)
  Interpreted MATLAB Function28/1 -> trans to column28/1(x)
  choose ksi_est_err 30/1(y) -> cal abs 30/1(x)
  Constant120/1 -> Mux27/2
  cal theta_sigma_bar_v_tilt agent 5/2(theta_sigma_bar_v_tilt_2_5) -> [theta_sigma_bar_v_tilt_2_5]
  [sigma_bar_v_tilt_vec] -> choose ksi_est_err 29/1(x)
  cal theta_sigma_bar_v_tilt agent 5/1(theta_sigma_bar_v_tilt_1_5) -> [theta_sigma_bar_v_tilt_1_5]
  [sigma_bar_v_tilt_vec] -> choose ksi_est_err 30/1(x)
  Constant119/1 -> Mux28/3
  trans to column28/1(y) -> [sigma_bar_v_tilt_squ_2_5], Display58/1
  Mux28/1 -> Interpreted MATLAB Function29/1
  Constant117/1 -> Mux28/2
  cal abs 29/1(y) -> Mux28/1
  [sigma_bar_v_tilt_squ_1_5] -> cal theta_sigma_bar_v_tilt agent 5/2(sigma_bar_v_tilt_squ_1_5)
  Mux27/1 -> Interpreted MATLAB Function28/1
  Constant121/1 -> Mux27/3
  Interpreted MATLAB Function29/1 -> trans to column29/1(x)
  [sigma_bar_v_tilt_vec] -> cal theta_sigma_bar_v_tilt agent 5/4(sigma_bar_v_tilt_vec)
  Constant118/1 -> cal theta_sigma_bar_v_tilt agent 5/1(alfa_theta)
  trans to column29/1(y) -> [sigma_bar_v_tilt_squ_1_5], Display59/1
  cal abs 30/1(y) -> Mux27/1
  combine theta_sigma_bar_v_tilt/1(theta_sigma_bar_v_tilt_1_vec) -> [theta_sigma_bar_v_tilt_1_vec]
  [theta_sigma_bar_v_tilt_2_1] -> combine theta_sigma_bar_v_tilt/6(theta_sigma_bar_v_tilt_2_1)
  [theta_sigma_bar_v_tilt_1_4] -> combine theta_sigma_bar_v_tilt/4(theta_sigma_bar_v_tilt_1_4)
  [theta_sigma_bar_v_tilt_2_2] -> combine theta_sigma_bar_v_tilt/7(theta_sigma_bar_v_tilt_2_2)
  [theta_sigma_bar_v_tilt_1_2] -> combine theta_sigma_bar_v_tilt/2(theta_sigma_bar_v_tilt_1_2)
  [theta_sigma_bar_v_tilt_2_5] -> combine theta_sigma_bar_v_tilt/10(theta_sigma_bar_v_tilt_2_5)
  [theta_sigma_bar_v_tilt_2_4] -> combine theta_sigma_bar_v_tilt/9(theta_sigma_bar_v_tilt_2_4)
  combine theta_sigma_bar_v_tilt/2(theta_sigma_bar_v_tilt_2_vec) -> [theta_sigma_bar_v_tilt_2_vec]
  [theta_sigma_bar_v_tilt_1_1] -> combine theta_sigma_bar_v_tilt/1(theta_sigma_bar_v_tilt_1_1)
  [theta_sigma_bar_v_tilt_2_3] -> combine theta_sigma_bar_v_tilt/8(theta_sigma_bar_v_tilt_2_3)
  [theta_sigma_bar_v_tilt_1_5] -> combine theta_sigma_bar_v_tilt/5(theta_sigma_bar_v_tilt_1_5)
  [theta_sigma_bar_v_tilt_1_3] -> combine theta_sigma_bar_v_tilt/3(theta_sigma_bar_v_tilt_1_3)
  Constant122/1 -> cal sigma_bar_v_hat agent 1/1(c1v)
  Constant123/1 -> cal sigma_bar_v_hat agent 1/2(c2v)
  [theta_sigma_bar_v_tilt_1_vec] -> cal sigma_bar_v_hat agent 1/3(theta_sigma_bar_v_tilt_1_vec)
  [theta_sigma_bar_v_tilt_2_vec] -> cal sigma_bar_v_hat agent 1/4(theta_sigma_bar_v_tilt_2_vec)
  [d_sigma_bar_v_vec] -> cal sigma_bar_v_hat agent 1/5(d_sigma_bar_v_vec)
  cal sigma_bar_v_hat agent 1/1(d_sigma_bar_v_hat_1) -> sigma_bar_v_hat Integrator 1/1
  [theta_sigma_bar_v_tilt_2_vec] -> cal sigma_bar_v_hat agent 2/4(theta_sigma_bar_v_tilt_2_vec)
  Constant125/1 -> cal sigma_bar_v_hat agent 2/2(c2v)
  cal sigma_bar_v_hat agent 2/1(d_sigma_bar_v_hat_2) -> sigma_bar_v_hat Integrator 2/1
  [d_sigma_bar_v_vec] -> cal sigma_bar_v_hat agent 2/5(d_sigma_bar_v_vec)
  [theta_sigma_bar_v_tilt_1_vec] -> cal sigma_bar_v_hat agent 2/3(theta_sigma_bar_v_tilt_1_vec)
  Constant124/1 -> cal sigma_bar_v_hat agent 2/1(c1v)
  Constant126/1 -> cal sigma_bar_v_hat agent 3/1(c1v)
  [theta_sigma_bar_v_tilt_2_vec] -> cal sigma_bar_v_hat agent 3/4(theta_sigma_bar_v_tilt_2_vec)
  cal sigma_bar_v_hat agent 3/1(d_sigma_bar_v_hat_3) -> sigma_bar_v_hat Integrator 3/1
  [d_sigma_bar_v_vec] -> cal sigma_bar_v_hat agent 3/5(d_sigma_bar_v_vec)
  Constant127/1 -> cal sigma_bar_v_hat agent 3/2(c2v)
  [theta_sigma_bar_v_tilt_1_vec] -> cal sigma_bar_v_hat agent 3/3(theta_sigma_bar_v_tilt_1_vec)
  [d_sigma_bar_v_vec] -> cal sigma_bar_v_hat agent 4/5(d_sigma_bar_v_vec)
  [theta_sigma_bar_v_tilt_1_vec] -> cal sigma_bar_v_hat agent 4/3(theta_sigma_bar_v_tilt_1_vec)
  Constant139/1 -> cal sigma_bar_v_hat agent 4/2(c2v)
  cal sigma_bar_v_hat agent 4/1(d_sigma_bar_v_hat_4) -> sigma_bar_v_hat Integrator 4/1
  [theta_sigma_bar_v_tilt_2_vec] -> cal sigma_bar_v_hat agent 4/4(theta_sigma_bar_v_tilt_2_vec)
  Constant128/1 -> cal sigma_bar_v_hat agent 4/1(c1v)
  [sigma_bar_v_hat_5] -> combine sigma_bar_v_hat/5(sigma_bar_v_hat_5)
  [sigma_bar_v_hat_4] -> combine sigma_bar_v_hat/4(sigma_bar_v_hat_4)
  [sigma_bar_v_hat_3] -> combine sigma_bar_v_hat/3(sigma_bar_v_hat_3)
  combine sigma_bar_v_hat/1(sigma_bar_v_hat_vec) -> [sigma_bar_v_hat_vec]
  cal combine sigma_bar_v_tilt/1(sigma_bar_v_tilt_vec) -> [sigma_bar_v_tilt_vec]
  [sigma_bar_v_vec] -> cal combine sigma_bar_v_tilt/1(sigma_bar_v_vec)
  [sigma_bar_v_hat_vec] -> cal combine sigma_bar_v_tilt/2(sigma_bar_v_hat_vec)
  [sigma_bar_v_hat_2] -> combine sigma_bar_v_hat/2(sigma_bar_v_hat_2)
  [sigma_bar_v_hat_1] -> combine sigma_bar_v_hat/1(sigma_bar_v_hat_1)
  sigma_bar_v_hat Integrator 1/1 -> [sigma_bar_v_hat_1]
  sigma_bar_v_hat Integrator 2/1 -> [sigma_bar_v_hat_2]
  sigma_bar_v_hat Integrator 3/1 -> [sigma_bar_v_hat_3]
  sigma_bar_v_hat Integrator 4/1 -> [sigma_bar_v_hat_4]
  sigma_bar_v_hat Integrator 5/1 -> [sigma_bar_v_hat_5]
  [d_sigma_bar_v_vec] -> cal sigma_bar_v_hat agent 5/5(d_sigma_bar_v_vec)
  [theta_sigma_bar_v_tilt_2_vec] -> cal sigma_bar_v_hat agent 5/4(theta_sigma_bar_v_tilt_2_vec)
  cal sigma_bar_v_hat agent 5/1(d_sigma_bar_v_hat_5) -> sigma_bar_v_hat Integrator 5/1
  [theta_sigma_bar_v_tilt_1_vec] -> cal sigma_bar_v_hat agent 5/3(theta_sigma_bar_v_tilt_1_vec)
  Constant141/1 -> cal sigma_bar_v_hat agent 5/2(c2v)
  Constant140/1 -> cal sigma_bar_v_hat agent 5/1(c1v)
  Constant142/1 -> cal dp_hat agent 1/1(c3v)
  [d_sigma_bar_v_vec] -> cal dp_hat agent 1/2(d_sigma_bar_v_vec)
  [sigma_bar_v_hat_vec] -> cal dp_hat agent 1/3(sigma_bar_v_hat_vec)
  cal dp_hat agent 1/1(dp_hat_1) -> [dp_hat_1]
  cal dp_hat agent 2/1(dp_hat_2) -> [dp_hat_2]
  [d_sigma_bar_v_vec] -> cal dp_hat agent 2/2(d_sigma_bar_v_vec)
  Constant143/1 -> cal dp_hat agent 2/1(c3v)
  [sigma_bar_v_hat_vec] -> cal dp_hat agent 2/3(sigma_bar_v_hat_vec)
  [sigma_bar_v_hat_vec] -> cal dp_hat agent 3/3(sigma_bar_v_hat_vec)
  Constant144/1 -> cal dp_hat agent 3/1(c3v)
  [d_sigma_bar_v_vec] -> cal dp_hat agent 3/2(d_sigma_bar_v_vec)
  cal dp_hat agent 3/1(dp_hat_3) -> [dp_hat_3]
  cal dp_hat agent 4/1(dp_hat_4) -> [dp_hat_4]
  [d_sigma_bar_v_vec] -> cal dp_hat agent 4/2(d_sigma_bar_v_vec)
  Constant145/1 -> cal dp_hat agent 4/1(c3v)
  [sigma_bar_v_hat_vec] -> cal dp_hat agent 4/3(sigma_bar_v_hat_vec)
  cal dp_hat agent 5/1(dp_hat_5) -> [dp_hat_5]
  [sigma_bar_v_hat_vec] -> cal dp_hat agent 5/3(sigma_bar_v_hat_vec)
  Constant146/1 -> cal dp_hat agent 5/1(c3v)
  [d_sigma_bar_v_vec] -> cal dp_hat agent 5/2(d_sigma_bar_v_vec)
  combine dp_hat/1(dp_hat_vec) -> [dp_hat_vec]
  [dp_hat_1] -> combine dp_hat/1(dp_hat_1)
  [dp_hat_4] -> combine dp_hat/4(dp_hat_4)
  [dp_hat_3] -> combine dp_hat/3(dp_hat_3)
  [dp_hat_5] -> combine dp_hat/5(dp_hat_5)
  [dp_hat_2] -> combine dp_hat/2(dp_hat_2)
  Constant148/1 -> cal theta_phi agent 1/1(alfa_theta)
  [phi_vec] -> cal theta_phi agent 1/4(phi_vec)
  [phi_squ_1_1] -> cal theta_phi agent 1/2(phi_squ_1_1)
  trans to column31/1(y) -> [phi_squ_1_1], Display61/1
  Interpreted MATLAB Function31/1 -> trans to column31/1(x)
  Mux31/1 -> Interpreted MATLAB Function31/1
  Constant151/1 -> Mux29/3
  cal theta_phi agent 1/1(theta_phi_1_1) -> [theta_phi_1_1]
  Constant147/1 -> Mux31/2
  trans to column30/1(y) -> [phi_squ_2_1], Display60/1
  Interpreted MATLAB Function30/1 -> trans to column30/1(x)
  cal abs 31/1(y) -> Mux31/1
  Constant149/1 -> Mux31/3
  Mux29/1 -> Interpreted MATLAB Function30/1
  choose ksi_est_err 32/1(y) -> cal abs 32/1(x)
  cal abs 32/1(y) -> Mux29/1
  choose ksi_est_err 31/1(y) -> cal abs 31/1(x)
  [phi_vec] -> choose ksi_est_err 32/1(x)
  [phi_squ_2_1] -> cal theta_phi agent 1/3(phi_squ_2_1)
  Constant150/1 -> Mux29/2
  [phi_vec] -> choose ksi_est_err 31/1(x)
  cal theta_phi agent 1/2(theta_phi_2_1) -> [theta_phi_2_1]
  cal theta_phi agent 2/2(theta_phi_2_2) -> [theta_phi_2_2]
  [phi_vec] -> choose ksi_est_err 33/1(x)
  [phi_squ_2_2] -> cal theta_phi agent 2/3(phi_squ_2_2)
  cal abs 34/1(y) -> Mux32/1
  choose ksi_est_err 34/1(y) -> cal abs 34/1(x)
  Constant154/1 -> Mux33/3
  Mux32/1 -> Interpreted MATLAB Function32/1
  Constant155/1 -> Mux32/2
  trans to column32/1(y) -> [phi_squ_2_2], Display62/1
  cal abs 33/1(y) -> Mux33/1
  [phi_vec] -> choose ksi_est_err 34/1(x)
  Interpreted MATLAB Function32/1 -> trans to column32/1(x)
  Constant152/1 -> Mux33/2
  cal theta_phi agent 2/1(theta_phi_1_2) -> [theta_phi_1_2]
  choose ksi_est_err 33/1(y) -> cal abs 33/1(x)
  [phi_squ_1_2] -> cal theta_phi agent 2/2(phi_squ_1_2)
  Interpreted MATLAB Function33/1 -> trans to column33/1(x)
  Constant156/1 -> Mux32/3
  [phi_vec] -> cal theta_phi agent 2/4(phi_vec)
  Mux33/1 -> Interpreted MATLAB Function33/1
  trans to column33/1(y) -> [phi_squ_1_2], Display63/1
  Constant153/1 -> cal theta_phi agent 2/1(alfa_theta)
  Constant158/1 -> cal theta_phi agent 3/1(alfa_theta)
  trans to column36/1(y) -> [phi_squ_1_3], Display70/1
  Interpreted MATLAB Function36/1 -> trans to column36/1(x)
  [phi_vec] -> cal theta_phi agent 3/4(phi_vec)
  [phi_squ_1_3] -> cal theta_phi agent 3/2(phi_squ_1_3)
  cal theta_phi agent 3/1(theta_phi_1_3) -> [theta_phi_1_3]
  choose ksi_est_err 35/1(y) -> cal abs 35/1(x)
  Mux35/1 -> Interpreted MATLAB Function36/1
  Constant161/1 -> Mux34/3
  [phi_vec] -> choose ksi_est_err 36/1(x)
  trans to column34/1(y) -> [phi_squ_2_3], Display69/1
  Interpreted MATLAB Function34/1 -> trans to column34/1(x)
  Constant157/1 -> Mux35/2
  cal abs 35/1(y) -> Mux35/1
  [phi_vec] -> choose ksi_est_err 35/1(x)
  choose ksi_est_err 36/1(y) -> cal abs 36/1(x)
  [phi_squ_2_3] -> cal theta_phi agent 3/3(phi_squ_2_3)
  Mux34/1 -> Interpreted MATLAB Function34/1
  Constant159/1 -> Mux35/3
  cal abs 36/1(y) -> Mux34/1
  cal theta_phi agent 3/2(theta_phi_2_3) -> [theta_phi_2_3]
  Constant160/1 -> Mux34/2
  choose ksi_est_err 38/1(y) -> cal abs 38/1(x)
  cal abs 37/1(y) -> Mux38/1
  [phi_vec] -> choose ksi_est_err 37/1(x)
  Mux37/1 -> Interpreted MATLAB Function37/1
  [phi_squ_2_4] -> cal theta_phi agent 4/3(phi_squ_2_4)
  Constant165/1 -> Mux37/2
  cal theta_phi agent 4/2(theta_phi_2_4) -> [theta_phi_2_4]
  cal abs 38/1(y) -> Mux37/1
  Interpreted MATLAB Function37/1 -> trans to column37/1(x)
  Constant164/1 -> Mux38/3
  [phi_vec] -> choose ksi_est_err 38/1(x)
  trans to column37/1(y) -> [phi_squ_2_4], Display71/1
  Constant162/1 -> Mux38/2
  [phi_vec] -> cal theta_phi agent 4/4(phi_vec)
  Mux38/1 -> Interpreted MATLAB Function38/1
  choose ksi_est_err 37/1(y) -> cal abs 37/1(x)
  Constant163/1 -> cal theta_phi agent 4/1(alfa_theta)
  Constant166/1 -> Mux37/3
  [phi_squ_1_4] -> cal theta_phi agent 4/2(phi_squ_1_4)
  cal theta_phi agent 4/1(theta_phi_1_4) -> [theta_phi_1_4]
  Interpreted MATLAB Function38/1 -> trans to column38/1(x)
  trans to column38/1(y) -> [phi_squ_1_4], Display72/1
  trans to column40/1(y) -> [phi_squ_1_5], Display75/1
  Interpreted MATLAB Function40/1 -> trans to column40/1(x)
  choose ksi_est_err 39/1(y) -> cal abs 39/1(x)
  Constant171/1 -> Mux39/3
  [phi_vec] -> cal theta_phi agent 5/4(phi_vec)
  [phi_squ_1_5] -> cal theta_phi agent 5/2(phi_squ_1_5)
  Constant168/1 -> cal theta_phi agent 5/1(alfa_theta)
  cal theta_phi agent 5/1(theta_phi_1_5) -> [theta_phi_1_5]
  Mux40/1 -> Interpreted MATLAB Function40/1
  Interpreted MATLAB Function39/1 -> trans to column39/1(x)
  Constant169/1 -> Mux40/3
  cal theta_phi agent 5/2(theta_phi_2_5) -> [theta_phi_2_5]
  Constant167/1 -> Mux40/2
  trans to column39/1(y) -> [phi_squ_2_5], Display73/1
  [phi_vec] -> choose ksi_est_err 40/1(x)
  [phi_vec] -> choose ksi_est_err 39/1(x)
  Mux39/1 -> Interpreted MATLAB Function39/1
  cal abs 40/1(y) -> Mux39/1
  choose ksi_est_err 40/1(y) -> cal abs 40/1(x)
  [phi_squ_2_5] -> cal theta_phi agent 5/3(phi_squ_2_5)
  cal abs 39/1(y) -> Mux40/1
  Constant170/1 -> Mux39/2
  combine theta_phi/1(theta_phi_1_vec) -> [theta_phi_1_vec]
  [theta_phi_2_1] -> combine theta_phi/6(theta_phi_2_1)
  [theta_phi_1_4] -> combine theta_phi/4(theta_phi_1_4)
  [theta_phi_2_2] -> combine theta_phi/7(theta_phi_2_2)
  [theta_phi_1_2] -> combine theta_phi/2(theta_phi_1_2)
  [theta_phi_2_5] -> combine theta_phi/10(theta_phi_2_5)
  [theta_phi_2_4] -> combine theta_phi/9(theta_phi_2_4)
  combine theta_phi/2(theta_phi_2_vec) -> [theta_phi_2_vec]
  [theta_phi_1_1] -> combine theta_phi/1(theta_phi_1_1)
  [theta_phi_2_3] -> combine theta_phi/8(theta_phi_2_3)
  [theta_phi_1_5] -> combine theta_phi/5(theta_phi_1_5)
  [theta_phi_1_3] -> combine theta_phi/3(theta_phi_1_3)
  Constant172/1 -> cal ui agent 1/1(kai_u_1)
  Constant173/1 -> cal ui agent 1/2(kai_u_2)
  [theta_phi_1_vec] -> cal ui agent 1/4(theta_phi_1_vec)
  [theta_phi_2_vec] -> cal ui agent 1/5(theta_phi_2_vec)
  [dp_hat_vec] -> cal ui agent 1/6(dp_hat_vec)
  cal ui agent 1/1(ui_1) -> [ui_1]
  [dp_hat_vec] -> cal ui agent 2/6(dp_hat_vec)
  Constant175/1 -> cal ui agent 2/2(kai_u_2)
  [theta_phi_1_vec] -> cal ui agent 2/4(theta_phi_1_vec)
  Constant174/1 -> cal ui agent 2/1(kai_u_1)
  cal ui agent 2/1(ui_2) -> [ui_2]
  [theta_phi_2_vec] -> cal ui agent 2/5(theta_phi_2_vec)
  [d_chi_vec] -> cal ui agent 2/3(d_chi_vec)
  [d_chi_vec] -> cal ui agent 3/3(d_chi_vec)
  [theta_phi_1_vec] -> cal ui agent 3/4(theta_phi_1_vec)
  [theta_phi_2_vec] -> cal ui agent 3/5(theta_phi_2_vec)
  cal ui agent 3/1(ui_3) -> [ui_3]
  Constant177/1 -> cal ui agent 3/2(kai_u_2)
  [dp_hat_vec] -> cal ui agent 3/6(dp_hat_vec)
  Constant176/1 -> cal ui agent 3/1(kai_u_1)
  [dp_hat_vec] -> cal ui agent 4/6(dp_hat_vec)
  Constant178/1 -> cal ui agent 4/1(kai_u_1)
  Constant179/1 -> cal ui agent 4/2(kai_u_2)
  [theta_phi_2_vec] -> cal ui agent 4/5(theta_phi_2_vec)
  [d_chi_vec] -> cal ui agent 4/3(d_chi_vec)
  [theta_phi_1_vec] -> cal ui agent 4/4(theta_phi_1_vec)
  cal ui agent 4/1(ui_4) -> [ui_4]
  [d_chi_vec] -> cal ui agent 5/3(d_chi_vec)
  [theta_phi_1_vec] -> cal ui agent 5/4(theta_phi_1_vec)
  [theta_phi_2_vec] -> cal ui agent 5/5(theta_phi_2_vec)
  Constant181/1 -> cal ui agent 5/2(kai_u_2)
  [dp_hat_vec] -> cal ui agent 5/6(dp_hat_vec)
  Constant180/1 -> cal ui agent 5/1(kai_u_1)
  cal ui agent 5/1(ui_5) -> [ui_5]
  [ui_5] -> combine ui/5(ui_5)
  [ui_2] -> combine ui/2(ui_2)
  [ui_1] -> combine ui/1(ui_1)
  [ui_4] -> combine ui/4(ui_4)
  [ui_3] -> combine ui/3(ui_3)
  [dp_vec] -> cal disturbance observation error dp_tilt/1(dp_vec)
  [dp_hat_vec] -> cal disturbance observation error dp_tilt/2(dp_hat_vec)
  cal disturbance observation error dp_tilt/1(dp_tilt_vec) -> [dp_tilt_vec]
  [dp_hat_vec] -> To Workspace1/1
  [dp_vec] -> To Workspace2/1
  [dp_tilt_vec] -> To Workspace6/1
  Demux11/2 -> dp_tilt_1/2
  Demux11/1 -> dp_tilt_1/1
  Demux11/3 -> dp_tilt_1/3
  choose dp_tilt_1/1(y) -> Demux11/1
  [dp_tilt_vec] -> choose dp_tilt_5/1(x), choose dp_tilt_4/1(x), choose dp_tilt_3/1(x), choose dp_tilt_2/1(x), choose dp_tilt_1/1(x)
  Demux13/1 -> dp_tilt_2/1
  Demux13/2 -> dp_tilt_2/2
  Demux13/3 -> dp_tilt_2/3
  choose dp_tilt_2/1(y) -> Demux13/1
  Demux14/3 -> dp_tilt_3/3
  Demux14/1 -> dp_tilt_3/1
  choose dp_tilt_3/1(y) -> Demux14/1
  Demux14/2 -> dp_tilt_3/2
  Demux15/1 -> dp_tilt_4/1
  choose dp_tilt_4/1(y) -> Demux15/1
  Demux15/2 -> dp_tilt_4/2
  Demux15/3 -> dp_tilt_4/3
  choose dp_tilt_5/1(y) -> Demux16/1
  Demux16/3 -> dp_tilt_5/3
  Demux16/1 -> dp_tilt_5/1
  Demux16/2 -> dp_tilt_5/2
  Demux17/1 -> sigma_bar_v_tilt_1/1
  Demux17/2 -> sigma_bar_v_tilt_1/2
  choose sigma_bar_v_tilt_1/1(y) -> Demux17/1
  Demux19/2 -> sigma_bar_v_tilt_3/2
  Demux19/1 -> sigma_bar_v_tilt_3/1
  choose sigma_bar_v_tilt_3/1(y) -> Demux19/1
  Demux19/3 -> sigma_bar_v_tilt_3/3
  Demux17/3 -> sigma_bar_v_tilt_1/3
  choose sigma_bar_v_tilt_5/1(y) -> Demux21/1
  Demux21/2 -> sigma_bar_v_tilt_5/2
  [sigma_bar_v_tilt_vec] -> choose sigma_bar_v_tilt_5/1(x), choose sigma_bar_v_tilt_4/1(x), choose sigma_bar_v_tilt_3/1(x), choose sigma_bar_v_tilt_2/1(x), choose sigma_bar_v_tilt_1/1(x)
  Demux21/1 -> sigma_bar_v_tilt_5/1
  Demux21/3 -> sigma_bar_v_tilt_5/3
  choose sigma_bar_v_tilt_4/1(y) -> Demux20/1
  Demux20/3 -> sigma_bar_v_tilt_4/3
  Demux20/2 -> sigma_bar_v_tilt_4/2
  Demux18/3 -> sigma_bar_v_tilt_2/3
  Demux20/1 -> sigma_bar_v_tilt_4/1
  Demux18/1 -> sigma_bar_v_tilt_2/1
  choose sigma_bar_v_tilt_2/1(y) -> Demux18/1
  Demux18/2 -> sigma_bar_v_tilt_2/2
  Demux34/2 -> phi_2/2
  Demux36/1 -> phi_4/1
  Demux34/3 -> phi_2/3
  Demux36/2 -> phi_4/2
  Demux36/3 -> phi_4/3
  choose phi_4/1(y) -> Demux36/1
  Demux37/3 -> phi_5/3
  Demux37/1 -> phi_5/1
  Demux35/3 -> phi_3/3
  Demux35/1 -> phi_3/1
  Demux34/1 -> phi_2/1
  choose phi_2/1(y) -> Demux34/1
  Demux35/2 -> phi_3/2
  Demux33/2 -> phi_1/2
  choose phi_1/1(y) -> Demux33/1
  choose phi_3/1(y) -> Demux35/1
  Demux33/1 -> phi_1/1
  [phi_vec] -> choose phi_5/1(x), choose phi_4/1(x), choose phi_3/1(x), choose phi_2/1(x), choose phi_1/1(x)
  Demux33/3 -> phi_1/3
  choose phi_5/1(y) -> Demux37/1
  Demux37/2 -> phi_5/2
  [sigma_bar_v_hat_vec] -> To Workspace11/1
  [sigma_bar_v_vec] -> To Workspace12/1
  [sigma_bar_v_tilt_vec] -> To Workspace13/1
  Demux38/3 -> Mux43/1
  Mux41/1 -> compare err_eta_1 and chi_1/1
  Mux43/1 -> compare err_eta_1 and chi_1/3
  Demux39/2 -> Mux42/2
  Demux39/3 -> Mux43/2
  Demux39/1 -> Mux41/2
  Demux38/2 -> Mux42/1
  Mux42/1 -> compare err_eta_1 and chi_1/2
  Demux38/1 -> Mux41/1
  choose err_eta_1/1(y) -> Demux39/1
  [err_eta_vec] -> choose err_eta_1/1(x)
  [chi_vec] -> choose chi_1/1(x)
  choose chi_1/1(y) -> Demux38/1
  choose chi_2/1(y) -> Demux40/1
  [chi_vec] -> choose chi_2/1(x)
  [err_eta_vec] -> choose err_eta_2/1(x)
  Mux45/1 -> compare err_eta_2 and chi_2/2
  Demux40/2 -> Mux45/1
  Demux41/1 -> Mux44/2
  Demux41/2 -> Mux45/2
  Mux46/1 -> compare err_eta_2 and chi_2/3
  choose err_eta_2/1(y) -> Demux41/1
  Mux44/1 -> compare err_eta_2 and chi_2/1
  Demux40/1 -> Mux44/1
  Demux40/3 -> Mux46/1
  Demux41/3 -> Mux46/2
  Demux43/3 -> Mux49/2
  Demux42/3 -> Mux49/1
  choose err_eta_3/1(y) -> Demux43/1
  Mux47/1 -> compare err_eta_3 and chi_3/1
  Mux49/1 -> compare err_eta_3 and chi_3/3
  [err_eta_vec] -> choose err_eta_3/1(x)
  Demux42/1 -> Mux47/1
  Demux43/1 -> Mux47/2
  Demux43/2 -> Mux48/2
  [chi_vec] -> choose chi_3/1(x)
  Mux48/1 -> compare err_eta_3 and chi_3/2
  Demux42/2 -> Mux48/1
  choose chi_3/1(y) -> Demux42/1
  [chi_vec] -> choose chi_4/1(x)
  choose chi_4/1(y) -> Demux44/1
  Demux44/2 -> Mux51/1
  Demux44/1 -> Mux50/1
  Demux45/2 -> Mux51/2
  Demux45/3 -> Mux52/2
  Mux51/1 -> compare err_eta_4 and chi_4/2
  Mux50/1 -> compare err_eta_4 and chi_4/1
  Mux52/1 -> compare err_eta_4 and chi_4/3
  Demux45/1 -> Mux50/2
  choose err_eta_4/1(y) -> Demux45/1
  Demux44/3 -> Mux52/1
  [err_eta_vec] -> choose err_eta_4/1(x)
  Demux46/3 -> Mux55/1
  [err_eta_vec] -> choose err_eta_5/1(x)
  Mux55/1 -> compare err_eta_5 and chi_5/3
  choose err_eta_5/1(y) -> Demux47/1
  Mux53/1 -> compare err_eta_5 and chi_5/1
  Demux47/1 -> Mux53/2
  Demux47/2 -> Mux54/2
  Demux46/2 -> Mux54/1
  Demux46/1 -> Mux53/1
  [chi_vec] -> choose chi_5/1(x)
  choose chi_5/1(y) -> Demux46/1
  Mux54/1 -> compare err_eta_5 and chi_5/2
  Demux47/3 -> Mux55/2
  choose sigma_bar_v_hat_1/1(y) -> Demux48/1
  Demux57/3 -> Mux70/2
  choose sigma_bar_v_hat_5/1(y) -> Demux56/1
  [sigma_bar_v_hat_vec] -> choose sigma_bar_v_hat_5/1(x)
  Demux57/2 -> Mux69/2
  choose sigma_bar_v_5/1(y) -> Demux57/1
  Demux56/3 -> Mux70/1
  Demux56/2 -> Mux69/1
  Mux70/1 -> compare sigma_bar_v_5 and sigma_bar_v_hat_5/3
  [sigma_bar_v_vec] -> choose sigma_bar_v_1/1(x)
  Mux57/1 -> compare sigma_bar_v_1 and sigma_bar_v_hat_1/2
  Demux49/3 -> Mux58/2
  Demux49/2 -> Mux57/2
  Demux48/3 -> Mux58/1
  Demux57/1 -> Mux68/2
  [sigma_bar_v_vec] -> choose sigma_bar_v_4/1(x)
  Demux56/1 -> Mux68/1
  [sigma_bar_v_hat_vec] -> choose sigma_bar_v_hat_1/1(x)
  Mux67/1 -> compare sigma_bar_v_4 and sigma_bar_v_hat_4/3
  Demux49/1 -> Mux56/2
  choose sigma_bar_v_4/1(y) -> Demux55/1
  Mux66/1 -> compare sigma_bar_v_4 and sigma_bar_v_hat_4/2
  Demux55/2 -> Mux66/2
  Demux54/2 -> Mux66/1
  Demux54/1 -> Mux65/1
  [sigma_bar_v_hat_vec] -> choose sigma_bar_v_hat_4/1(x)
  [sigma_bar_v_hat_vec] -> choose sigma_bar_v_hat_3/1(x)
  Demux54/3 -> Mux67/1
  Mux63/1 -> compare sigma_bar_v_3 and sigma_bar_v_hat_3/2
  [sigma_bar_v_vec] -> choose sigma_bar_v_5/1(x)
  Demux52/1 -> Mux62/1
  [sigma_bar_v_vec] -> choose sigma_bar_v_3/1(x)
  Demux53/2 -> Mux63/2
  Demux53/3 -> Mux64/2
  Mux65/1 -> compare sigma_bar_v_4 and sigma_bar_v_hat_4/1
  Mux62/1 -> compare sigma_bar_v_3 and sigma_bar_v_hat_3/1
  Mux64/1 -> compare sigma_bar_v_3 and sigma_bar_v_hat_3/3
  Demux52/3 -> Mux64/1
  Demux55/3 -> Mux67/2
  Mux56/1 -> compare sigma_bar_v_1 and sigma_bar_v_hat_1/1
  Demux51/3 -> Mux61/2
  Demux52/2 -> Mux63/1
  Demux50/3 -> Mux61/1
  choose sigma_bar_v_2/1(y) -> Demux51/1
  Demux48/2 -> Mux57/1
  Demux55/1 -> Mux65/2
  Mux59/1 -> compare sigma_bar_v_2 and sigma_bar_v_hat_2/1
  Mux61/1 -> compare sigma_bar_v_2 and sigma_bar_v_hat_2/3
  [sigma_bar_v_vec] -> choose sigma_bar_v_2/1(x)
  Mux68/1 -> compare sigma_bar_v_5 and sigma_bar_v_hat_5/1
  choose sigma_bar_v_1/1(y) -> Demux49/1
  Demux53/1 -> Mux62/2
  Demux50/1 -> Mux59/1
  Mux58/1 -> compare sigma_bar_v_1 and sigma_bar_v_hat_1/3
  Demux51/1 -> Mux59/2
  choose sigma_bar_v_hat_3/1(y) -> Demux52/1
  Mux69/1 -> compare sigma_bar_v_5 and sigma_bar_v_hat_5/2
  Demux51/2 -> Mux60/2
  choose sigma_bar_v_hat_4/1(y) -> Demux54/1
  Demux48/1 -> Mux56/1
  [sigma_bar_v_hat_vec] -> choose sigma_bar_v_hat_2/1(x)
  Mux60/1 -> compare sigma_bar_v_2 and sigma_bar_v_hat_2/2
  Demux50/2 -> Mux60/1
  choose sigma_bar_v_hat_2/1(y) -> Demux50/1
  choose sigma_bar_v_3/1(y) -> Demux53/1
  choose dp_1/1(y) -> Demux59/1
  Demux61/1 -> Mux74/2
  Mux83/1 -> compare dp_5 and dp_hat_5/1
  Demux58/2 -> Mux72/1
  [dp_vec] -> choose dp_2/1(x)
  Mux76/1 -> compare dp_2 and dp_hat_2/3
  Mux71/1 -> compare dp_1 and dp_hat_1/1
  Demux62/3 -> Mux79/1
  Mux79/1 -> compare dp_3 and dp_hat_3/3
  Demux61/3 -> Mux76/2
  Demux62/2 -> Mux78/1
  Mux77/1 -> compare dp_3 and dp_hat_3/1
  Demux65/3 -> Mux82/2
  [dp_vec] -> choose dp_3/1(x)
  Mux80/1 -> compare dp_4 and dp_hat_4/1
  Demux60/3 -> Mux76/1
  Mux73/1 -> compare dp_1 and dp_hat_1/3
  Demux63/1 -> Mux77/2
  Demux63/3 -> Mux79/2
  Demux63/2 -> Mux78/2
  Demux64/3 -> Mux82/1
  Demux62/1 -> Mux77/1
  Mux78/1 -> compare dp_3 and dp_hat_3/2
  [dp_vec] -> choose dp_5/1(x)
  [dp_hat_vec] -> choose dp_hat_3/1(x)
  [dp_hat_vec] -> choose dp_hat_4/1(x)
  Demux64/1 -> Mux80/1
  Demux64/2 -> Mux81/1
  Demux65/2 -> Mux81/2
  Demux65/1 -> Mux80/2
  Demux59/1 -> Mux71/2
  Demux60/1 -> Mux74/1
  choose dp_4/1(y) -> Demux65/1
  Mux81/1 -> compare dp_4 and dp_hat_4/2
  Demux67/1 -> Mux83/2
  choose dp_2/1(y) -> Demux61/1
  [dp_hat_vec] -> choose dp_hat_1/1(x)
  Demux59/2 -> Mux72/2
  [dp_vec] -> choose dp_4/1(x)
  choose dp_hat_3/1(y) -> Demux62/1
  Mux82/1 -> compare dp_4 and dp_hat_4/3
  Mux72/1 -> compare dp_1 and dp_hat_1/2
  Demux59/3 -> Mux73/2
  [dp_vec] -> choose dp_1/1(x)
  Mux74/1 -> compare dp_2 and dp_hat_2/1
  Mux85/1 -> compare dp_5 and dp_hat_5/3
  Demux66/3 -> Mux85/1
  choose dp_5/1(y) -> Demux67/1
  Demux66/2 -> Mux84/1
  choose dp_hat_1/1(y) -> Demux58/1
  choose dp_hat_5/1(y) -> Demux66/1
  Mux84/1 -> compare dp_5 and dp_hat_5/2
  choose dp_3/1(y) -> Demux63/1
  Demux67/3 -> Mux85/2
  Demux66/1 -> Mux83/1
  Demux61/2 -> Mux75/2
  choose dp_hat_2/1(y) -> Demux60/1
  Mux75/1 -> compare dp_2 and dp_hat_2/2
  Demux58/1 -> Mux71/1
  [dp_hat_vec] -> choose dp_hat_2/1(x)
  Demux67/2 -> Mux84/2
  Demux60/2 -> Mux75/1
  choose dp_hat_4/1(y) -> Demux64/1
  [dp_hat_vec] -> choose dp_hat_5/1(x)
  Demux58/3 -> Mux73/1
  [phi_vec] -> To Workspace16/1
  [chi_vec] -> To Workspace15/1
  Constant280/1 -> Mux129/3
  Mux128/1 -> Interpreted MATLAB Function50/1
  choose eta_est_err_tilt 13/1(y) -> cal abs 45/1(x)
  choose eta_est_err_tilt 12/1(y) -> cal abs 44/1(x)
  [ksi_est_err_tilt_vec] -> choose eta_est_err_tilt 14/1(x)
  cal abs 48/1(y) -> Mux124/1
  trans to column46/1(y) -> [ksi_est_err_squ_2_node_3], Display80/1
  [eta_est_err_tilt_vec] -> choose eta_est_err_tilt 10/1(x)
  Constant247/1 -> Mux109/2
  [ksi0] -> cal lumped observation error agent 2/4(ksi0)
  [theta_eta_est_err_tilt_1_vec] -> fixed-time distributed follower desire velocity observer agent 2/3(theta_eta_est_err_tilt_1_vec)
  Interpreted MATLAB Function47/1 -> trans to column47/1(x)
  Constant273/1 -> Mux123/3
  Constant227/1 -> cal lumped observation error agent 2/1(wij)
  Interpreted MATLAB Function46/1 -> trans to column46/1(x)
  choose eta_est_err_tilt 15/1(y) -> cal abs 47/1(x)
  choose eta_est_err_tilt 5/1(y) -> cal abs 56/1(x)
  choose eta_est_err_tilt 14/1(y) -> cal abs 46/1(x)
  cal abs 43/1(y) -> Mux126/1
  Constant218/1 -> Mux120/3
  choose eta_est_err_tilt 16/1(y) -> cal abs 48/1(x)
  Constant220/1 -> Mux122/2
  trans to column45/1(y) -> [ksi_est_err_squ_1_node_1], Display84/1
  Constant200/1 -> fixed-time distributed follower desire velocity observer agent 1/1(l1v)
  Constant281/1 -> Mux128/2
  Constant214/1 -> Add4/2
  Interpreted MATLAB Function50/1 -> trans to column50/1(x)
  Add3/1 -> Demux76/1
  trans to column50/1(y) -> [ksi_est_err_squ_2_node_5], Display85/1
  cal theta_ksi_est_err_tilt agent 1/1(theta_ksi_est_err_tilt_1_1) -> [theta_ksi_est_err_tilt_1_1]
  [eta_est_err_squ_1_node_3] -> cal theta_eta_est_err_tilt agent 3/2(eta_est_err_squ_1_node_3)
  Add8/1 -> Demux97/1
  [eta_est_err_squ_1_node_2] -> cal theta_eta_est_err_tilt agent 2/2(eta_est_err_squ_1_node_2)
  Constant263/1 -> fixed-time distributed follower desire position observer agent 3/1(l1p)
  Mux134/1 -> ksi_d_est_3/2
  cal theta_ksi_est_err_tilt agent 5/2(theta_ksi_est_err_tilt_2_5) -> [theta_ksi_est_err_tilt_2_5]
  [eta_d_est_vec] -> fixed-time distributed follower desire position observer agent 1/3(eta_d_est_vec)
  Interpreted MATLAB Function56/1 -> trans to column56/1(x)
  cal theta_ksi_est_err_tilt agent 2/2(theta_ksi_est_err_tilt_2_2) -> [theta_ksi_est_err_tilt_2_2]
  Constant248/1 -> Mux109/3
  Constant252/1 -> fixed-time distributed follower desire position observer agent 3/2(l2p)
  Mux135/1 -> ksi_d_est_3/3
  trans to column48/1(y) -> [ksi_est_err_squ_2_node_4], Display82/1
  Demux93/2 -> Mux130/2
  [theta_eta_est_err_tilt_2_3] -> combine lumped follower velocity observation error/8(theta_eta_est_err_tilt_2_3)
  [theta_eta_est_err_tilt_1_3] -> combine lumped follower velocity observation error/3(theta_eta_est_err_tilt_1_3)
  position observe Integrator 2/1 -> [ksi_d_est_2], Demux92/1
  Demux95/3 -> Mux135/2
  [ksi0] -> cal lumped observation error agent 1/4(ksi0)
  Demux94/2 -> Mux134/1
  [theta_eta_est_err_tilt_2_vec] -> fixed-time distributed follower desire velocity observer agent 5/4(theta_eta_est_err_tilt_2_vec)
  Mux109/1 -> Interpreted MATLAB Function41/1
  [ksi0] -> Add6/1
  velocity observe Integrator 5/1 -> [eta_d_est_5], Demux77/1
  Constant268/1 -> Mux121/2
  Demux93/1 -> Mux119/2
  fixed-time distributed follower desire position observer agent 2/1(d_ksi_d_est_2) -> position observe Integrator 2/1
  Demux93/3 -> Mux132/2
  [theta_ksi_est_err_tilt_1_vec] -> fixed-time distributed follower desire position observer agent 3/4(theta_ksi_est_err_tilt_1_vec)
  [ksi_est_err_squ_1_node_3] -> cal theta_ksi_est_err_tilt agent 3/2(ksi_est_err_squ_1_node_3)
  Constant216/1 -> Mux126/3
  Mux108/1 -> ksi_d_est_1/3
  trans to column43/1(y) -> [ksi_est_err_squ_2_node_2], Display78/1
  Mux113/1 -> Interpreted MATLAB Function56/1
  [ksi_est_err_tilt_vec] -> choose eta_est_err_tilt 18/1(x)
  Add6/1 -> Demux93/1
  Mux119/1 -> ksi_d_est_2/1
  [theta_eta_est_err_tilt_1_1] -> combine lumped follower velocity observation error/1(theta_eta_est_err_tilt_1_1)
  Interpreted MATLAB Function53/1 -> trans to column53/1(x)
  cal theta_eta_est_err_tilt agent 3/1(theta_eta_est_err_tilt_1_3) -> [theta_eta_est_err_tilt_1_3]
  Demux88/3 -> Mux108/2
  Demux88/1 -> Mux86/2
  Add5/1 -> Demux88/1
  [eta_est_err_tilt_3] -> "combine lumped follower observation error "/8(eta_est_err_tilt_3)
  Constant261/1 -> Mux114/3
  Constant270/1 -> Mux124/2
  Demux73/2 -> Mux100/1
  Constant267/1 -> Mux122/3
  cal abs 60/1(y) -> Mux118/1
  [theta_ksi_est_err_tilt_1_3] -> combine lumped follower position observation error/3(theta_ksi_est_err_tilt_1_3)
  [theta_ksi_est_err_tilt_2_4] -> combine lumped follower position observation error/9(theta_ksi_est_err_tilt_2_4)
  Mux117/1 -> Interpreted MATLAB Function59/1
  cal theta_ksi_est_err_tilt agent 4/2(theta_ksi_est_err_tilt_2_4) -> [theta_ksi_est_err_tilt_2_4]
  trans to column47/1(y) -> [ksi_est_err_squ_1_node_3], Display81/1
  Add1/1 -> Demux72/1
  [ksi0] -> cal lumped observation error agent 3/4(ksi0)
  Constant203/1 -> fixed-time distributed follower desire velocity observer agent 2/1(l1v)
  cal abs 44/1(y) -> Mux128/1
  [eta_d_est_vec] -> cal lumped observation error agent 1/6(eta_d_est_vec)
  Mux127/1 -> Interpreted MATLAB Function49/1
  Constant278/1 -> Mux125/3
  [theta_eta_est_err_tilt_1_vec] -> fixed-time distributed follower desire velocity observer agent 5/3(theta_eta_est_err_tilt_1_vec)
  [ksi_est_err_tilt_4] -> "combine lumped follower observation error "/4(ksi_est_err_tilt_4)
  [ksi_est_err_tilt_vec] -> choose eta_est_err_tilt 12/1(x)
  trans to column51/1(y) -> [ksi_est_err_squ_1_node_5], Display86/1
  Interpreted MATLAB Function51/1 -> trans to column51/1(x)
  trans to column56/1(y) -> [eta_est_err_squ_1_node_3], Display90/1
  choose eta_est_err_tilt 18/1(y) -> cal abs 50/1(x)
  [ksi_est_err_tilt_vec] -> cal theta_ksi_est_err_tilt agent 1/4(ksi_est_err_tilt_vec)
  Mux103/1 -> eta_d_est_4/2
  velocity observe Integrator 4/1 -> [eta_d_est_4], Demux75/1
  Demux77/2 -> Mux106/1
  Demux77/1 -> Mux105/1
  Mux107/1 -> eta_d_est_5/3
  fixed-time distributed follower desire velocity observer agent 5/1(d_eta_d_est_5) -> velocity observe Integrator 5/1
  [theta_eta_est_err_tilt_2_5] -> combine lumped follower velocity observation error/10(theta_eta_est_err_tilt_2_5)
  Mux104/1 -> eta_d_est_4/3
  Demux74/3 -> Mux101/2
  Constant205/1 -> fixed-time distributed follower desire velocity observer agent 3/2(l2v)
  fixed-time distributed follower desire velocity observer agent 3/1(d_eta_d_est_3) -> velocity observe Integrator 3/1
  Demux74/2 -> Mux100/2
  Demux75/2 -> Mux103/1
  Constant207/1 -> Add2/2
  Demux76/3 -> Mux104/2
  Demux75/3 -> Mux104/1
  cal lumped observation error agent 4/2(eta_est_err_tilt_4) -> [eta_est_err_tilt_4]
  Mux95/1 -> eta_d_est_2/1
  velocity observe Integrator 3/1 -> [eta_d_est_3], Demux73/1
  velocity observe Integrator 2/1 -> [eta_d_est_2], Demux71/1
  Demux72/1 -> Mux95/2
  [eta0] -> Add2/1
  [eta_est_err_tilt_5] -> "combine lumped follower observation error "/10(eta_est_err_tilt_5)
  cal abs 45/1(y) -> Mux120/1
  Add/1 -> Demux70/1
  cal lumped observation error agent 2/1(ksi_est_err_tilt_2) -> [ksi_est_err_tilt_2]
  cal theta_eta_est_err_tilt agent 5/2(theta_eta_est_err_tilt_2_5) -> [theta_eta_est_err_tilt_2_5]
  fixed-time distributed follower desire velocity observer agent 2/1(d_eta_d_est_2) -> velocity observe Integrator 2/1
  [theta_eta_est_err_tilt_2_vec] -> fixed-time distributed follower desire velocity observer agent 2/4(theta_eta_est_err_tilt_2_vec)
  Mux98/1 -> eta_d_est_2/3
  [eta_est_err_tilt_vec] -> cal theta_eta_est_err_tilt agent 4/4(eta_est_err_tilt_vec)
  [eta_d_est_5] -> combine follower desire velocity estimaters/5(eta_d_est_5)
  trans to column60/1(y) -> [eta_est_err_squ_1_node_5], Display95/1
  cal lumped observation error agent 3/1(ksi_est_err_tilt_3) -> [ksi_est_err_tilt_3]
  [eta_est_err_squ_2_node_2] -> cal theta_eta_est_err_tilt agent 2/3(eta_est_err_squ_2_node_2)
  cal theta_eta_est_err_tilt agent 3/2(theta_eta_est_err_tilt_2_3) -> [theta_eta_est_err_tilt_2_3]
  cal theta_eta_est_err_tilt agent 1/2(theta_eta_est_err_tilt_2_1) -> [theta_eta_est_err_tilt_2_1]
  [eta_est_err_tilt_vec] -> cal theta_eta_est_err_tilt agent 2/4(eta_est_err_tilt_vec)
  [eta_est_err_squ_1_node_4] -> cal theta_eta_est_err_tilt agent 4/2(eta_est_err_squ_1_node_4)
  cal theta_eta_est_err_tilt agent 2/2(theta_eta_est_err_tilt_2_2) -> [theta_eta_est_err_tilt_2_2]
  [eta_est_err_tilt_vec] -> choose eta_est_err_tilt 9/1(x)
  Demux72/2 -> Mux96/2
  [theta_eta_est_err_tilt_2_1] -> combine lumped follower velocity observation error/6(theta_eta_est_err_tilt_2_1)
  [eta_est_err_tilt_vec] -> choose eta_est_err_tilt 5/1(x)
  [eta_est_err_tilt_vec] -> cal theta_eta_est_err_tilt agent 1/4(eta_est_err_tilt_vec)
  choose eta_est_err_tilt 10/1(y) -> cal abs 42/1(x)
  [eta_est_err_squ_1_node_1] -> cal theta_eta_est_err_tilt agent 1/2(eta_est_err_squ_1_node_1)
  [theta_eta_est_err_tilt_1_4] -> combine lumped follower velocity observation error/4(theta_eta_est_err_tilt_1_4)
  [theta_ksi_est_err_tilt_2_5] -> combine lumped follower position observation error/10(theta_ksi_est_err_tilt_2_5)
  Constant259/1 -> Mux116/3
  choose eta_est_err_tilt 4/1(y) -> cal abs 55/1(x)
  choose eta_est_err_tilt 8/1(y) -> cal abs 59/1(x)
  Mux118/1 -> Interpreted MATLAB Function60/1
  Constant266/1 -> Mux117/3
  Constant262/1 -> Mux118/2
  Constant255/1 -> Mux113/3
  [eta_est_err_tilt_vec] -> choose eta_est_err_tilt 7/1(x)
  [ksi_d_est_vec] -> cal lumped observation error agent 5/3(ksi_d_est_vec)
  Interpreted MATLAB Function58/1 -> trans to column58/1(x)
  [eta_d_est_2] -> combine follower desire velocity estimaters/2(eta_d_est_2)
  Mux114/1 -> Interpreted MATLAB Function57/1
  cal abs 59/1(y) -> Mux114/1
  Constant260/1 -> Mux114/2
  Interpreted MATLAB Function55/1 -> trans to column55/1(x)
  trans to column58/1(y) -> [eta_est_err_squ_1_node_4], Display92/1
  Constant228/1 -> cal lumped observation error agent 2/2(w0)
  [theta_ksi_est_err_tilt_2_1] -> combine lumped follower position observation error/6(theta_ksi_est_err_tilt_2_1)
  Constant249/1 -> Mux111/2
  Constant265/1 -> Mux117/2
  cal abs 51/1(y) -> Mux125/1
  Mux112/1 -> Interpreted MATLAB Function55/1
  Mux111/1 -> Interpreted MATLAB Function53/1
  Constant250/1 -> Mux111/3
  cal theta_eta_est_err_tilt agent 5/1(theta_eta_est_err_tilt_1_5) -> [theta_eta_est_err_tilt_1_5]
  choose eta_est_err_tilt 3/1(y) -> cal abs 54/1(x)
  trans to column52/1(y) -> [eta_est_err_squ_2_node_2], Display87/1
  [ksi_est_err_tilt_2] -> "combine lumped follower observation error "/2(ksi_est_err_tilt_2)
  cal abs 42/1(y) -> Mux117/1
  Constant254/1 -> Mux113/2
  Constant256/1 -> Mux112/2
  [ksi_est_err_tilt_5] -> "combine lumped follower observation error "/5(ksi_est_err_tilt_5)
  Demux76/1 -> Mux102/2
  [theta_eta_est_err_tilt_1_5] -> combine lumped follower velocity observation error/5(theta_eta_est_err_tilt_1_5)
  choose eta_est_err_tilt 1/1(y) -> cal abs 41/1(x)
  choose eta_est_err_tilt 9/1(y) -> cal abs 60/1(x)
  Mux110/1 -> Interpreted MATLAB Function52/1
  Constant251/1 -> Mux110/2
  Mux124/1 -> Interpreted MATLAB Function47/1
  cal lumped observation error agent 5/1(ksi_est_err_tilt_5) -> [ksi_est_err_tilt_5]
  [eta_est_err_tilt_2] -> "combine lumped follower observation error "/7(eta_est_err_tilt_2)
  Mux123/1 -> Interpreted MATLAB Function46/1
  [ksi_d_est_vec] -> cal lumped observation error agent 3/3(ksi_d_est_vec)
  Constant242/1 -> cal lumped observation error agent 5/2(w0)
  [ksi_d_est_vec] -> cal lumped observation error agent 4/3(ksi_d_est_vec)
  Mux105/1 -> eta_d_est_5/1
  [ksi_est_err_squ_2_node_1] -> cal theta_ksi_est_err_tilt agent 1/3(ksi_est_err_squ_2_node_1)
  [eta_est_err_tilt_4] -> "combine lumped follower observation error "/9(eta_est_err_tilt_4)
  Add7/1 -> Demux95/1
  Constant217/1 -> Mux120/2
  Constant236/1 -> cal lumped observation error agent 4/1(wij)
  [eta0] -> cal lumped observation error agent 1/7(eta0)
  [eta0] -> cal lumped observation error agent 2/7(eta0)
  choose eta_est_err_tilt 17/1(y) -> cal abs 49/1(x)
  cal lumped observation error agent 1/2(eta_est_err_tilt_1) -> [eta_est_err_tilt_1]
  Demux77/3 -> Mux107/1
  cal lumped observation error agent 1/1(ksi_est_err_tilt_1) -> [ksi_est_err_tilt_1]
  trans to column44/1(y) -> [ksi_est_err_squ_1_node_2], Display79/1
  [eta_d_est_vec] -> cal lumped observation error agent 2/6(eta_d_est_vec)
  cal lumped observation error agent 4/1(ksi_est_err_tilt_4) -> [ksi_est_err_tilt_4]
